simulink model "GFo_29bus"  (R2020b)
settings: Solver=ode1  StartTime=0.0  StopTime=4.5  FixedStep=Time_Step  RelTol=1e-3  EnableMultiTasking=on
PreLoadFcn:
  | Init_29bus;
InitFcn:
  | Init_29bus;
undefined symbols (not defined in the file): D1, D11, Delta, Time_Step, VSC01_Delta_P_Time_Step, VSC01_Delta_P_Value
libraries: powerlib x169, sps_avr x6, GFo_Lib x1
(part 2 of 5)

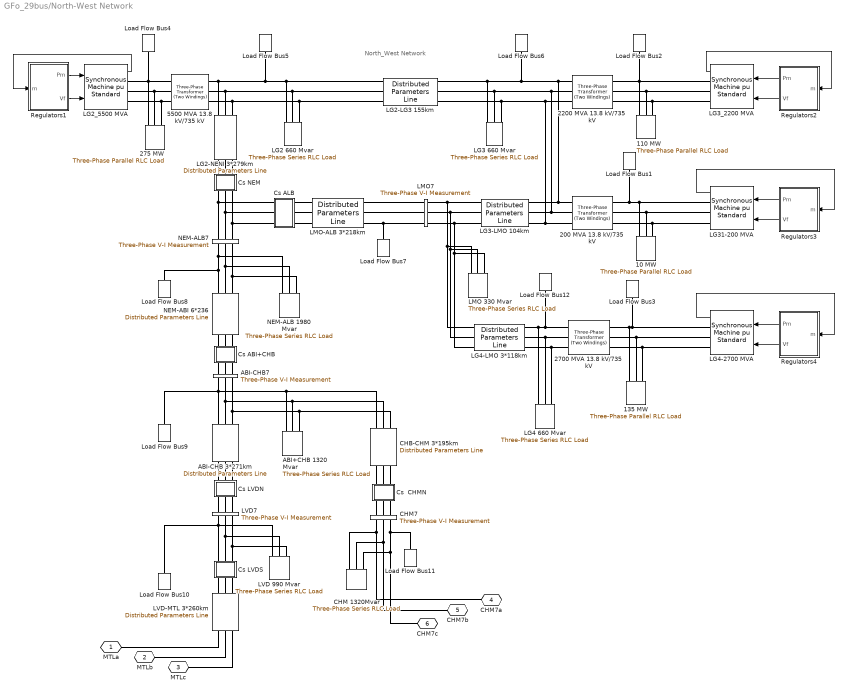
== system GFo_29bus/North-West Network ==
  note: North_West Network
  10 MW : powerlib/Elements/Three-Phase Parallel RLC Load  LConnTagsString=A|B|C  Configuration=Y (grounded)  NominalVoltage=(13800)*1  Vabc=[1e3 1e3 1e3]  Vabcp=[1e3 1e3 1e3]  NominalFrequency=60  UnbalancedPower=off  ActivePower=10000000  InductivePower=0  CapacitivePower=0  Pabc=[10e3 9e3 11e3]  QLabc=[100 90 110]  QCabc=[100 90 110]  Pabcp=[10e3 9e3 11e3]  QLabcp=[100 90 110]  QCabcp=[100 90 110]  Measurements=None  LoadType=constant PQ
  110 MW : powerlib/Elements/Three-Phase Parallel RLC Load  LConnTagsString=A|B|C  Configuration=Y (grounded)  NominalVoltage=(13800)*1  Vabc=[1e3 1e3 1e3]  Vabcp=[1e3 1e3 1e3]  NominalFrequency=60  UnbalancedPower=off  ActivePower=110000000  InductivePower=0  CapacitivePower=0  Pabc=[10e3 9e3 11e3]  QLabc=[100 90 110]  QCabc=[100 90 110]  Pabcp=[10e3 9e3 11e3]  QLabcp=[100 90 110]  QCabcp=[100 90 110]  Measurements=None  LoadType=constant PQ
  135 MW : powerlib/Elements/Three-Phase Parallel RLC Load  LConnTagsString=A|B|C  Configuration=Y (grounded)  NominalVoltage=(13800)*1  Vabc=[1e3 1e3 1e3]  Vabcp=[1e3 1e3 1e3]  NominalFrequency=60  UnbalancedPower=off  ActivePower=135000000  InductivePower=0  CapacitivePower=0  Pabc=[10e3 9e3 11e3]  QLabc=[100 90 110]  QCabc=[100 90 110]  Pabcp=[10e3 9e3 11e3]  QLabcp=[100 90 110]  QCabcp=[100 90 110]  Measurements=None  LoadType=constant PQ
  200 MVA 13.8 kV/735 kV : powerlib/Elements/Three-Phase Transformer (Two Windings)  Winding1Connection=Delta (D1)  Winding2Connection=Yg  CoreType=Three single-phase transformers  SetSaturation=off  Hysteresis=off  DataFile='basic_model'  SetInitialFlux=off  Measurements=None  UNITS=pu  NominalPower=[ 200e6 60 ]  Winding1="[ 13.8e3 0.002  0.0]"  Winding2=[ 735e3 0.002 0.12]  Rm=500  Lm=500  L0=0.5  Saturation="[ 0,0  ;  0.005,1.2  ;  1.0,1.4 ]"  InitialFluxes=[ 0.8 , -0.8 , 0.7 ]  BreakLoop=off  DiscreteSolver=Trapezoidal iterative  DataType=off  TransfoNumber=0
  2200 MVA 13.8 kV/735 kV : powerlib/Elements/Three-Phase Transformer (Two Windings)  Winding1Connection=Delta (D1)  Winding2Connection=Yg  CoreType=Three single-phase transformers  SetSaturation=off  Hysteresis=off  DataFile='basic_model'  SetInitialFlux=off  Measurements=None  UNITS=pu  NominalPower=[ 2200e6 60 ]  Winding1="[ 13.8e3 0.002  0.0]"  Winding2=[ 735e3 0.002 0.12]  Rm=500  Lm=500  L0=0.5  Saturation="[ 0,0  ;  0.005,1.2  ;  1.0,1.4 ]"  InitialFluxes=[ 0.8 , -0.8 , 0.7 ]  BreakLoop=off  DiscreteSolver=Trapezoidal iterative  DataType=off  TransfoNumber=0
  2700 MVA 13.8 kV/735 kV : powerlib/Elements/Three-Phase Transformer (Two Windings)  Winding1Connection=Delta (D1)  Winding2Connection=Yg  CoreType=Three single-phase transformers  SetSaturation=off  Hysteresis=off  DataFile='basic_model'  SetInitialFlux=off  Measurements=None  UNITS=pu  NominalPower=[ 2700e6 60 ]  Winding1="[ 13.8e3 0.002  0.0]"  Winding2=[ 735e3 0.002 0.12]  Rm=500  Lm=500  L0=0.5  Saturation="[ 0,0  ;  0.005,1.2  ;  1.0,1.4 ]"  InitialFluxes=[ 0.8 , -0.8 , 0.7 ]  BreakLoop=off  DiscreteSolver=Trapezoidal iterative  DataType=off  TransfoNumber=0
  275 MW : powerlib/Elements/Three-Phase Parallel RLC Load  LConnTagsString=A|B|C  Configuration=Y (grounded)  NominalVoltage=(13800)*1  Vabc=[1e3 1e3 1e3]  Vabcp=[1e3 1e3 1e3]  NominalFrequency=60  UnbalancedPower=off  ActivePower=275000000  InductivePower=0  CapacitivePower=0  Pabc=[10e3 9e3 11e3]  QLabc=[100 90 110]  QCabc=[100 90 110]  Pabcp=[10e3 9e3 11e3]  QLabcp=[100 90 110]  QCabcp=[100 90 110]  Measurements=None  LoadType=constant PQ
  5500 MVA 13.8 kV/735 kV : powerlib/Elements/Three-Phase Transformer (Two Windings)  Winding1Connection=Delta (D1)  Winding2Connection=Yg  CoreType=Three single-phase transformers  SetSaturation=off  Hysteresis=off  DataFile='basic_model'  SetInitialFlux=off  Measurements=None  UNITS=pu  NominalPower=[ 5500e6 60 ]  Winding1="[ 13.8e3 0.002  0.0]"  Winding2=[ 735e3 0.002 0.12]  Rm=500  Lm=500  L0=0.5  Saturation="[ 0,0  ;  0.005,1.2  ;  1.0,1.4 ]"  InitialFluxes=[ 0.8 , -0.8 , 0.7 ]  BreakLoop=off  DiscreteSolver=Trapezoidal iterative  DataType=off  TransfoNumber=0
  ABI+CHB 1320 Mvar : powerlib/Elements/Three-Phase Series RLC Load  LConnTagsString=A|B|C  Configuration=Y (grounded)  NominalVoltage=735e3  Vabc=[1e3 1e3 1e3]  Vabcp=[1e3 1e3 1e3]  NominalFrequency=60  UnbalancedPower=off  ActivePower=4400000  InductivePower=1320e6  CapacitivePower=0  Pabc=[10e3 9e3 11e3]  QLabc=[100 90 110]  QCabc=[100 90 110]  Pabcp=[10e3 9e3 11e3]  QLabcp=[100 90 110]  QCabcp=[100 90 110]  Measurements=None  LoadType=constant Z
  ABI-CHB 3*271km : powerlib/Elements/Distributed Parameters Line  Phases=3  Length=271  Frequency=60  Resistance="[0.01273  0.3864]/3"  Inductance="[0.9337e-3  4.1264e-3]/3"  Capacitance=[12.74e-9 7.751e-9]*3  x1=[-0.00156 1.39752875491723e-07 0 0;-0.00152 1.40446452432915e-07 0 0;-0.00148 1.41108093061983e-07 0 0;-0.00144 1.41737646927554e-07 0 0;-0.0014 1.42334970874506e-07 0 0;-0.00136 1.42899929076526e-07 0 0;-0.00132 1.4343239306699e-07 0 0;-0.00128 1.43932241768179e-07 0 0;-0.00124 1.44399361518809e-07 0 0;-0.0012 1.44833646099877e-07 0 0;-0.00116 1.45234996758813e-07 0 0;-0.00112 1.4560332223194e-07 0 0;-0.00108 1.45938538765221e-07 0 0;-0.00104 1.46240570133307e-07 0 0;-0.001 1.4650934765687e-07 0 0;-0.00096 1.46744810218219e-07 187826.147215716 -755236.018624843;-0.00092 1.46946904275197e-07 199193.07837809 -752317.887921003;-0.00088 1.47115583873359e-07 210514.71475221 -749228.686617163;-0.00084 1.47250810656419e-07 221788.481895596 -745969.11717106;-0.0008 1.47352553874973e-07 233011.816250821 -742539.920780675;-0.00076 1.4742079039349e-07 244182.16572844 -738941.877215697;-0.00072 1.47455504695574e-07 255296.990287309 -735175.804640203;-0.00068 1.47456688887492e-07 266353.762512174 -731242.55942662;-0.00064 1.4742434269997e-07 277349.968188381 -727143.035960991;-0.0006 1.47358473488251e-07 288283.106873586 -722878.166439598;-0.00056 1.47259096230426e-07 299150.692466336 -718448.920656993;-0.00052 1.47126233524027e-07 309950.253771385 -713856.305785471;-0.00048 1.46959915580887e-07 320679.335061623 -709101.366146047;-0.00044 1.46760180220273e-07 331335.496636489 -704185.182970991;-0.0004 1.46527072860282e-07 341916.315376735 -699108.874157963;-0.00036 1.46260646507518e-07 352419.385295425 -693873.594015808;-0.00032 1.45960961745037e-07 362842.318085035 -688480.533002086;-0.00028 1.45628086718568e-07 373182.743660531 -682930.917452362;-0.00024 1.45262097121023e-07 383438.31069831 -677226.009301355;-0.0002 1.4486307617528e-07 393606.687170866 -671367.105795981;-0.00016 1.4443111461526e-07 403685.56087708 -665355.539200373;-0.00012 1.43966310665298e-07 413672.639967986 -659192.676492932;-8e-05 1.43468770017803e-07 423565.653467925 -652879.919055492;-4e-05 1.42938605809227e-07 433362.351790939 -646418.702354656]  x2=[-0.00156 2.99200739443898e-07 0 0;-0.00152 3.00668696195938e-07 0 0;-0.00148 3.02068283479319e-07 0 0;-0.00144 3.03399183039963e-07 0 0;-0.0014 3.04661092242786e-07 0 0;-0.00136 3.05853724140519e-07 0 0;-0.00132 3.06976807538953e-07 0 0;-0.00128 3.08030087058607e-07 0 0;-0.00124 3.09013323192803e-07 0 0;-0.0012 3.09926292362122e-07 0 0;-0.00116 3.10768786965248e-07 0 0;-0.00112 3.11540615426174e-07 0 0;-0.00108 3.12241602237765e-07 0 0;-0.00104 3.12871588001663e-07 0 0;-0.001 3.13430429464539e-07 0 0;-0.00096 3.13917999550664e-07 -41952.3785136554 -761003.958677179;-0.00092 3.14334187390805e-07 -30472.3572707285 -761550.015312884;-0.00088 3.14678898347436e-07 -18985.4068765407 -761922.902042434;-0.00084 3.14952054036257e-07 -7494.13936455236 -762122.534074602;-0.0008 3.15153592344022e-07 3998.83225010076 -762148.866014787;-0.00076 3.15283467442656e-07 15490.8945647847 -762001.891875332;-0.00072 3.15341649799683e-07 26979.4343836324 -761681.64507689;-0.00068 3.15328126184936e-07 38461.839311762 -761188.198440819;-0.00064 3.15242899673569e-07 49935.4983493129 -760521.664172631;-0.0006 3.15085989645354e-07 61397.8024851645 -759682.193836469;-0.00056 3.14857431780281e-07 72846.1452902031 -758669.978320649;-0.00052 3.14557278050435e-07 84277.9235100011 -757485.24779425;-0.00048 3.14185596708187e-07 95690.5376567748 -756128.271654777;-0.00044 3.13742472270669e-07 107081.392600485 -754599.358466902;-0.0004 3.13228005500556e-07 118447.898158949 -752898.8558923;-0.00036 3.12642313383155e-07 129787.469686823 -751027.150610591;-0.00032 3.11985529099804e-07 141097.528663329 -748984.668231415;-0.00028 3.11257801997584e-07 152375.503278591 -746771.873197653;-0.00024 3.10459297555363e-07 163618.829018437 -744389.268679811;-0.0002 3.09590197346165e-07 174824.949247554 -741837.396461612;-0.00016 3.08650698995882e-07 185991.315790837 -739116.83681679;-0.00012 3.07641016138338e-07 197115.389512831 -736228.208377148;-8e-05 3.06561378366707e-07 208194.6408951 -733172.167991883;-4e-05 3.05412031181309e-07 219226.550611423 -729949.410578225]  x3=[-0.00156 3.57527130254717e-10 0 0;-0.00152 3.79613404300157e-10 0 0;-0.00148 4.01613357531105e-10 0 0;-0.00144 4.23521987347916e-10 0 0;-0.0014 4.45334311917103e-10 0 0;-0.00136 4.67045371304159e-10 0 0;-0.00132 4.88650228601409e-10 0 0;-0.00128 5.10143971050614e-10 0 0;-0.00124 5.31521711160097e-10 0 0;-0.0012 5.5277858781611e-10 0 0;-0.00116 5.73909767388214e-10 0 0;-0.00112 5.949104448284e-10 0 0;-0.00108 6.15775844763721e-10 0 0;-0.00104 6.36501222582168e-10 0 0;-0.001 6.57081865511553e-10 0 0;-0.00096 6.77513093691153e-10 139.261704598099 -1341.51413254979;-0.00092 6.97790261235871e-10 159.474777333089 -1339.26171711188;-0.00088 7.17908757292671e-10 179.651586878967 -1336.7047651088;-0.00084 7.37864007089045e-10 199.787545203237 -1333.84385796939;-0.0008 7.57651472973275e-10 219.878073562622 -1330.67964623925;-0.00076 7.77266655446258e-10 239.918603544227 -1327.21284943285;-0.00072 7.96705094184655e-10 259.904578104356 -1323.44425586989;-0.00068 8.15962369055127e-10 279.831452604746 -1319.37472249604;-0.00064 8.35034101119436e-10 299.694695845977 -1315.00517468809;-0.0006 8.53915953630177e-10 319.48979109783 -1310.33660604355;-0.00056 8.7260363301692e-10 339.212237126349 -1305.37007815465;-0.00052 8.91092889862529e-10 358.857549217388 -1300.10672036701;-0.00048 9.0937951986944e-10 378.42126019639 -1294.5477295228;-0.00044 9.27459364815689e-10 397.89892144419 -1288.6943696886;-0.0004 9.45328313500447e-10 417.286103908588 -1282.54797186797;-0.00036 9.62982302678879e-10 436.578399111478 -1276.10993369875;-0.00032 9.80417317986088e-10 455.771420151303 -1269.38171913531;-0.00028 9.97629394849945e-10 474.860802700591 -1262.36485811562;-0.00024 1.0146146193926e-09 493.842205998369 -1255.06094621337;-0.0002 1.03136912932048e-09 512.711313837218 -1247.47164427514;-0.00016 1.04788911480249e-09 531.463835544733 -1239.59867804273;-0.00012 1.06417081933641e-09 550.095506959195 -1231.44383776078;-8e-05 1.08021054060303e-09 568.602091399196 -1223.00897776964;-4e-05 1.09600463130805e-09 586.979380627029 -1214.29601608374]  x4=[-0.00156 1.09221564098943e-09 0 0;-0.00152 1.08563764232773e-09 0 0;-0.00148 1.07881277902829e-09 0 0;-0.00144 1.0717426030062e-09 0 0;-0.0014 1.06442872195849e-09 0 0;-0.00136 1.05687279899865e-09 0 0;-0.00132 1.0490765522784e-09 0 0;-0.00128 1.04104175459702e-09 0 0;-0.00124 1.0327702329982e-09 0 0;-0.0012 1.02426386835463e-09 0 0;-0.00116 1.01552459494027e-09 0 0;-0.00112 1.00655439999053e-09 0 0;-0.00108 9.97355323250386e-10 0 0;-0.00104 9.87929456510564e-10 0 0;-0.001 9.78278943131873e-10 0 0;-0.00096 9.68405977557831e-10 -1510.55195138334 -15585.3803111024;-0.00092 9.58312804815671e-10 -1275.36683491454 -15606.3854409047;-0.00088 9.48001720005832e-10 -1039.89171102577 -15623.8418132415;-0.00084 9.37475067780084e-10 -804.180124729557 -15637.7454586843;-0.0008 9.26735241808363e-10 -568.285674807936 -15648.0932156639;-0.00076 9.15784684234478e-10 -332.262001624548 -15654.8827311897;-0.00072 9.0462588512079e-10 -96.1627749272983 -15658.1124613844;-0.00068 8.93261381881987e-10 139.958318355698 -15657.7816718352;-0.00064 8.81693758708102e-10 376.04758632405 -15653.8904377607;-0.0006 8.69925645976889e-10 612.051344314168 -15646.4396439941;-0.00056 8.57959719655701e-10 847.915927106694 -15635.4309847816;-0.00052 8.45798700692993e-10 1083.58770112951 -15620.8669633974;-0.00048 8.33445354399604e-10 1319.01307665356 -15602.7508915744;-0.00044 8.20902489819951e-10 1554.13851997865 -15581.0868887509;-0.0004 8.08172959093275e-10 1788.91056560663 -15555.8798811346;-0.00036 7.95259656805089e-10 2023.27582839889 -15527.1356005815;-0.00032 7.82165519328971e-10 2257.18101571576 -15494.8605832931;-0.00028 7.68893524158867e-10 2490.57293953476 -15459.0621683301;-0.00024 7.55446689232024e-10 2723.39852854509 -15419.7484959432;-0.0002 7.41828072242744e-10 2955.60484021562 -15376.9285057226;-0.00016 7.2804076994709e-10 3187.13907283354 -15330.6119345649;-0.00012 7.14087917458705e-10 3417.94857751101 -15280.8093144587;-8e-05 6.99972687535923e-10 3647.98087015709 -15227.5319700906;-4e-05 6.85698289860302e-10 3877.18364341214 -15170.792016269]  x5=0.00153261764655846  V1=ones(3,3)  V2=ones(3,3)  I1=ones(3,3)  I2=ones(3,3)  nHarmo=1  Measurements=None  Decoupling=off  VsMag0=0  VrMag0=0  VsAngle0=0  VrAngle0=0  IsMag0=0  IrMag0=0  IsAngle0=0  IrAngle0=0
      settings: AttributesFormatString=\n
  ABI-CHB7 : powerlib/Measurements/Three-Phase V-I Measurement  VoltageMeasurement=no  SetLabelV=on  LabelV=Vabc_ABI7  Vpu=on  VpuLL=off  CurrentMeasurement=no  SetLabelI=off  LabelI=A1  Ipu=off  Pbase=100e6  Vbase=500e3  OutputType=Magnitude  PhasorSimulation=off  PSBequivalent=0
  CHB-CHM 3*195km : powerlib/Elements/Distributed Parameters Line  Phases=3  Length=195  Frequency=60  Resistance="[0.01273  0.3864]/3"  Inductance="[0.9337e-3  4.1264e-3]/3"  Capacitance=[12.74e-9 7.751e-9]*3  x1=[-0.00112 1.45810315855676e-07 0 0;-0.00108 1.46144986641095e-07 0 0;-0.00104 1.46446425316851e-07 0 0;-0.001 1.46714563338391e-07 0 0;-0.00096 1.4694933973344e-07 0 0;-0.00092 1.47150701115871e-07 0 0;-0.00088 1.47318601697842e-07 0 0;-0.00084 1.47453003300208e-07 0 0;-0.0008 1.47553875361205e-07 0 0;-0.00076 1.47621194943394e-07 0 0;-0.00072 1.47654946738885e-07 0 0;-0.00068 1.47655123072809e-07 266353.762512174 -731242.55942662;-0.00064 1.4762172390507e-07 277349.968188381 -727143.035960991;-0.0006 1.4755475683035e-07 288283.106873586 -722878.166439599;-0.00056 1.47454237076385e-07 299150.692466336 -718448.920656994;-0.00052 1.473201875005e-07 309950.253771385 -713856.305785471;-0.00048 1.47152638584413e-07 320679.335061623 -709101.366146047;-0.00044 1.46951628427302e-07 331335.496636489 -704185.182970992;-0.0004 1.46717202737144e-07 341916.315376735 -699108.874157963;-0.00036 1.46449414820318e-07 352419.385295425 -693873.594015809;-0.00032 1.46148325569488e-07 362842.318085035 -688480.533002086;-0.00028 1.45814003449753e-07 373182.743660531 -682930.917452362;-0.00024 1.4544652448308e-07 383438.31069831 -677226.009301355;-0.0002 1.45045972231017e-07 393606.687170866 -671367.105795982;-0.00016 1.44612437775692e-07 403685.56087708 -665355.539200373;-0.00012 1.44146019699101e-07 413672.639967986 -659192.676492932;-8e-05 1.43646824060693e-07 423565.653467925 -652879.919055493;-4e-05 1.43114964373251e-07 433362.351790939 -646418.702354656]  x2=[-0.00112 1.02653671848885e-07 0 0;-0.00108 1.02818285588003e-07 0 0;-0.00104 1.02959519335645e-07 0 0;-0.001 1.03077340976476e-07 0 0;-0.00096 1.03171723718869e-07 0 0;-0.00092 1.03242646101004e-07 0 0;-0.00088 1.03290091995742e-07 0 0;-0.00084 1.03314050614296e-07 0 0;-0.0008 1.03314516508683e-07 0 0;-0.00076 1.03291489572962e-07 0 0;-0.00072 1.0324497504326e-07 0 0;-0.00068 1.03174983496581e-07 189059.279163622 -739106.876621779;-0.00064 1.03081530848397e-07 200182.85637729 -736171.980405194;-0.0006 1.02964638349035e-07 211260.913735721 -733069.685028741;-0.00056 1.02824332578842e-07 222290.932184205 -729800.695927637;-0.00052 1.0266064544214e-07 233270.403591666 -726365.756441812;-0.00048 1.02473614159972e-07 244196.831320988 -722765.647646883;-0.00044 1.02263281261639e-07 255067.730796732 -719001.188176545;-0.0004 1.02029694575028e-07 265880.630070103 -715073.234036418;-0.00036 1.01772907215738e-07 276633.070381053 -710982.6784094;-0.00032 1.01492977574998e-07 287322.60671738 -706730.451452565;-0.00028 1.01189969306396e-07 297946.808370705 -702317.520085654;-0.00024 1.00863951311399e-07 308503.25948919 -697744.887771204;-0.0002 1.00514997723688e-07 318989.559626885 -693013.59428637;-0.00016 1.00143187892299e-07 329403.324289571 -688124.71548649;-0.00012 9.97486063635805e-08 339742.185476966 -683079.363060443;-8e-05 9.93313428619707e-08 350003.792221196 -677878.684277862;-4e-05 9.88914922695912e-08 360185.811121378 -672523.861728252]  x3=[-0.00112 5.46806558992984e-10 0 0;-0.00108 5.43566628750611e-10 0 0;-0.00104 5.40203096144379e-10 0 0;-0.001 5.36716726012596e-10 0 0;-0.00096 5.33108311125766e-10 0 0;-0.00092 5.29378672006317e-10 0 0;-0.00088 5.2552865674202e-10 0 0;-0.00084 5.21559140793147e-10 0 0;-0.0008 5.17471026793391e-10 0 0;-0.00076 5.13265244344623e-10 0 0;-0.00072 5.08942749805502e-10 0 0;-0.00068 5.0450452607401e-10 1436.68883540451 -5039.58498648989;-0.00064 4.99951582363951e-10 1512.51770856541 -5017.34797480586;-0.0006 4.95284953975461e-10 1588.00264824277 -4993.97006146011;-0.00056 4.90505702059593e-10 1663.12648981228 -4969.45656238856;-0.00052 4.85614913377017e-10 1737.87215076019 -4943.81305174949;-0.00048 4.80613700050904e-10 1812.2226345678 -4917.04536065607;-0.00044 4.75503199314036e-10 1886.16103457624 -4889.15957585044;-0.0004 4.70284573250208e-10 1959.67053783099 -4860.16203831958;-0.00036 4.64959008529985e-10 2032.7344289049 -4830.05934185345;-0.00032 4.59527716140858e-10 2105.33609369925 -4798.85833154564;-0.00028 4.53991931111878e-10 2177.45902322152 -4766.56610223683;-0.00024 4.48352912232824e-10 2249.08681733953 -4733.18999690149;-0.0002 4.42611941767958e-10 2320.20318851057 -4698.73760497815;-0.00016 4.36770325164458e-10 2390.79196548512 -4663.21676064362;-0.00012 4.30829390755561e-10 2460.83709698404 -4626.63554103159;-8e-05 4.24790489458522e-10 2530.32265534845 -4589.00226439593;-4e-05 4.18654994467416e-10 2599.23284016162 -4550.32548821922]  x4=[-0.00112 3.66592185990391e-10 0 0;-0.00108 3.74745086886299e-10 0 0;-0.00104 3.82812773981113e-10 0 0;-0.001 3.90793412752361e-10 0 0;-0.00096 3.98685188471607e-10 0 0;-0.00092 4.0648630661711e-10 0 0;-0.00088 4.14194993281876e-10 0 0;-0.00084 4.21809495577036e-10 0 0;-0.0008 4.29328082030432e-10 0 0;-0.00076 4.36749042980341e-10 0 0;-0.00072 4.44070690964241e-10 0 0;-0.00068 4.51291361102517e-10 1508.00651437075 -11782.2938614844;-0.00064 4.5840941147705e-10 1685.50172841415 -11758.2144968013;-0.0006 4.65423223504567e-10 1862.61367389965 -11731.4614155401;-0.00056 4.72331202304699e-10 2039.3020770982 -11702.0407011208;-0.00052 4.79131777062637e-10 2215.52676059061 -11669.9590435602;-0.00048 4.85823401386327e-10 2391.24765240356 -11635.2237379506;-0.00044 4.92404553658105e-10 2566.42479512158 -11597.8426828008;-0.0004 4.98873737380697e-10 2741.01835497311 -11557.8243782405;-0.00036 5.05229481517512e-10 2914.98863088824 -11515.177924087;-0.00032 5.11470340827144e-10 3088.29606352651 -11469.9130177763;-0.00028 5.17594896192004e-10 3260.90124427226 -11422.0399521576;-0.00024 5.23601754941019e-10 3432.76492419587 -11371.5696131533;-0.0002 5.29489551166309e-10 3603.84802297863 -11318.5134772832;-0.00016 5.35256946033787e-10 3774.11163779923 -11262.883609055;-0.00012 5.40902628087596e-10 3943.51705217994 -11204.6926582211;-8e-05 5.46425313548324e-10 4112.02574479043 -11143.9538569019;-4e-05 5.51823746604922e-10 4279.59939820715 -11080.681016577]  x5=0.0011028060556417  V1=ones(3,3)  V2=ones(3,3)  I1=ones(3,3)  I2=ones(3,3)  nHarmo=1  Measurements=None  Decoupling=off  VsMag0=0  VrMag0=0  VsAngle0=0  VrAngle0=0  IsMag0=0  IrMag0=0  IsAngle0=0  IrAngle0=0
      settings: AttributesFormatString=\n
  CHM 1320Mvar : powerlib/Elements/Three-Phase Series RLC Load  LConnTagsString=A|B|C  Configuration=Y (grounded)  NominalVoltage=735e3  Vabc=[1e3 1e3 1e3]  Vabcp=[1e3 1e3 1e3]  NominalFrequency=60  UnbalancedPower=off  ActivePower=4400000  InductivePower=1320e6  CapacitivePower=0  Pabc=[10e3 9e3 11e3]  QLabc=[100 90 110]  QCabc=[100 90 110]  Pabcp=[10e3 9e3 11e3]  QLabcp=[100 90 110]  QCabcp=[100 90 110]  Measurements=None  LoadType=constant Z
  CHM7 : powerlib/Measurements/Three-Phase V-I Measurement  VoltageMeasurement=no  SetLabelV=on  LabelV=Vabc_CHM7  Vpu=on  VpuLL=off  CurrentMeasurement=no  SetLabelI=off  LabelI=A1  Ipu=off  Pbase=100e6  Vbase=735e3  OutputType=Magnitude  PhasorSimulation=off  PSBequivalent=0
  "Cs  CHMN " : Subsystem  mask{Xc=25/3}
      mask prompts: Xc "Condensator Reactance at  60Hz  (ohm):"
      mask help: Series Compensation
      mask init:
      | Cs=1/Xc/(2*pi*60);
      mask Display: disp('Cs')
  "Cs ABI+CHB " : Subsystem  mask{Xc=25/6}
      mask prompts: Xc "Condensator Reactance at  60Hz  (ohm):"
      mask help: Series Compensation
      mask init:
      | Cs=1/Xc/(2*pi*60);
      mask Display: disp('Cs')
  Cs ALB : Subsystem  mask{Xc=16/3}
      mask prompts: Xc "Reactance @ 60Hz du condensateur (ohm):"
      mask init:
      | Cs=1/Xc/(2*pi*60);
      mask Display: disp('Cs')
  "Cs LVDN " : Subsystem  mask{Xc=34/3}
      mask prompts: Xc "Condensator Reactance at  60Hz  (ohm):"
      mask help: Series Compensation
      mask init:
      | Cs=1/Xc/(2*pi*60);
      mask Display: disp('Cs')
  "Cs LVDS " : Subsystem  mask{Xc=34/3}
      mask prompts: Xc "Condensator Reactance at  60Hz  (ohm):"
      mask help: Series Compensation
      mask init:
      | Cs=1/Xc/(2*pi*60);
      mask Display: disp('Cs')
  "Cs NEM " : Subsystem  mask{Xc=16/3}
      mask prompts: Xc "Condensator Reactance at  60Hz  (ohm):"
      mask help: Series Compensation
      mask init:
      | Cs=1/Xc/(2*pi*60);
      mask Display: disp('Cs')
  LG2 660 Mvar : powerlib/Elements/Three-Phase Series RLC Load  LConnTagsString=A|B|C  Configuration=Y (grounded)  NominalVoltage=735e3  Vabc=[1e3 1e3 1e3]  Vabcp=[1e3 1e3 1e3]  NominalFrequency=60  UnbalancedPower=off  ActivePower=2200000  InductivePower=660e6  CapacitivePower=0  Pabc=[10e3 9e3 11e3]  QLabc=[100 90 110]  QCabc=[100 90 110]  Pabcp=[10e3 9e3 11e3]  QLabcp=[100 90 110]  QCabcp=[100 90 110]  Measurements=None  LoadType=constant Z
  LG2-LG3 155km : powerlib/Elements/Distributed Parameters Line  Phases=3  Length=155  Frequency=60  Resistance="[0.01273  0.3864]"  Inductance="[0.9337e-3  4.1264e-3]"  Capacitance=[12.74e-9 7.751e-9]  x1=[-0.00088 8.27904700189463e-09 432972.643007168 -601762.460463716;-0.00084 8.1824988858554e-09 441997.469609916 -595165.210790078;-0.0008 8.08409014013239e-09 450921.789799698 -588432.625679992;-0.00076 7.98384314202574e-09 459743.574263063 -581566.236065254;-0.00072 7.88178068683832e-09 468460.817002301 -574567.603303648;-0.00068 7.7779259826923e-09 477071.535791587 -567438.318823911;-0.00064 7.67230264525179e-09 485573.772627723 -560180.003763853;-0.0006 7.56493469235287e-09 493965.594175373 -552794.308601725;-0.00056 7.45584653854213e-09 502245.092206687 -545282.912780917;-0.00052 7.345062989525e-09 510410.384035209 -537647.524328061;-0.00048 7.23260923652519e-09 518459.612943993 -529889.879464649;-0.00044 7.11851085055635e-09 526390.9486078 -522011.742212222;-0.0004 7.00279377660752e-09 534202.587509295 -514014.903991253;-0.00036 6.88548432774341e-09 541892.753349157 -505901.183213792;-0.00032 6.76660917912106e-09 549459.697449992 -497672.424869975;-0.00028 6.64619536192413e-09 556901.699153965 -489330.500108486;-0.00024 6.52427025721625e-09 564217.066214066 -480877.305811079;-0.0002 6.40086158971478e-09 571404.135178912 -472314.76416124;-0.00016 6.27599742148649e-09 578461.271770996 -463644.8222071;-0.00012 6.14970614556646e-09 585386.871258318 -454869.451418693;-8e-05 6.02201647950173e-09 592179.358819277 -445990.64723966;-4e-05 5.89295745882122e-09 598837.189900778 -437010.428633504]  x2=[-0.00088 2.7409355673421e-09 445028.999861563 -584528.468417923;-0.00084 2.64624629672137e-09 453792.581408512 -577751.376045215;-0.0008 2.55095529251302e-09 462452.97443579 -570842.90799191;-0.00076 2.45508422306966e-09 471008.209644705 -563804.635184068;-0.00072 2.35865488864571e-09 479456.341648548 -556638.158064228;-0.00068 2.26168921644027e-09 487795.449414957 -549345.106227488;-0.00064 2.16420925561097e-09 496023.636702737 -541927.138050943;-0.0006 2.0662371722603e-09 504139.032493056 -534385.940316585;-0.00056 1.96779524439513e-09 512139.791414897 -526723.227827747;-0.00052 1.86890585686093e-09 520024.094164675 -518940.743019169;-0.00048 1.76959149625163e-09 527790.147919937 -511040.255560782;-0.00044 1.66987474579639e-09 535436.18674703 -503023.561955305;-0.0004 1.56977828022435e-09 542960.472002662 -494892.485129729;-0.00036 1.46932486060857e-09 550361.292729253 -486648.874020806;-0.00032 1.36853732919041e-09 557636.96604399 -478294.603154611;-0.00028 1.26743860418535e-09 564785.837521505 -469831.572220297;-0.00024 1.16605167457163e-09 571806.281570074 -461261.705638114;-0.0002 1.06439959486271e-09 578696.701801261 -452586.952121821;-0.00016 9.62505479864911e-10 585455.531392926 -443809.284235559;-0.00012 8.60392499421284e-10 592081.233445506 -434930.69794531;-8e-05 7.58083873142997e-10 598572.301331491 -425953.21216503;-4e-05 6.55602865129395e-10 604927.259038022 -416878.868297569]  x3=[-0.00088 7.27991996063612e-12 1691.0601492433 -2581.83555988018;-0.00084 6.86444585434417e-12 1729.79962719017 -2556.0423915541;-0.0008 6.44741083226141e-12 1768.14576361897 -2529.66800123056;-0.00076 6.02890972455549e-12 1806.08983894897 -2502.71838621846;-0.00072 5.60903769476932e-12 1843.62322502464 -2475.19967462786;-0.00068 5.18789021818163e-12 1880.73738707768 -2447.11812397646;-0.00064 4.76556306009679e-12 1917.42388566768 -2418.48011976672;-0.0006 4.34215225406855e-12 1953.67437860124 -2389.29217403383;-0.00056 3.91775408006286e-12 1989.48062282887 -2359.56092386494;-0.00052 3.49246504256463e-12 2024.83447631943 -2329.29312988995;-0.00048 3.06638184863347e-12 2059.7278999115 -2298.49567474419;-0.00044 2.63960138591327e-12 2094.15295914146 -2267.17556150338;-0.0004 2.21222070060087e-12 2128.10182604773 -2235.33991209117;-0.00036 1.78433697537853e-12 2161.56678095071 -2202.99596565971;-0.00032 1.35604750731546e-12 2194.54021420827 -2170.15107694348;-0.00028 9.2744968574328e-13 2227.01462794603 -2136.81271458693;-0.00024 4.98640970110547e-13 2258.98263776235 -2102.98845944618;-0.0002 6.97188678213079e-14 2290.43697440747 -2068.68600286516;-0.00016 -3.59219087937244e-13 2321.37048543651 -2033.91314492666;-0.00012 -7.88075360372972e-13 2351.7761368358 -1998.67779267874;-8e-05 -1.21675243126782e-12 2381.64701462243 -1962.98795833662;-4e-05 -1.64515282315263e-12 2410.97632641638 -1926.85175746086]  x4=[-0.00088 1.00066401297176e-11 1092.96989342867 -2102.93040181918;-0.00084 1.02141033117926e-11 1124.5560468815 -2086.21026082815;-0.0008 1.04192438948573e-11 1155.88648598704 -2069.01573361452;-0.00076 1.06220152317119e-11 1186.95408647359 -2051.35073006549;-0.00072 1.08223712139033e-11 1217.75178383675 -2033.21926705055;-0.00068 1.10202662822087e-11 1248.2725749457 -2014.62546750801;-0.00064 1.12156554369963e-11 1278.50951963575 -1995.57355950756;-0.0006 1.14084942484572e-11 1308.45574228643 -1976.06787528876;-0.00056 1.15987388667087e-11 1338.10443338496 -1956.11285027601;-0.00052 1.17863460317652e-11 1367.44885107466 -1935.7130220699;-0.00048 1.19712730833751e-11 1396.482322688 -1914.87302941546;-0.00044 1.21534779707218e-11 1425.19824626391 -1893.59761114728;-0.0004 1.2332919261985e-11 1453.59009204901 -1871.89160511202;-0.00036 1.25095561537627e-11 1481.6514039824 -1849.75994706827;-0.00032 1.26833484803488e-11 1509.37580116375 -1827.2076695642;-0.00028 1.2854256722867e-11 1536.75697930421 -1804.23990079324;-0.00024 1.30222420182568e-11 1563.78871216001 -1780.86186342794;-0.0002 1.31872661681107e-11 1590.4648529482 -1757.0788734324;-0.00016 1.33492916473601e-11 1616.77933574442 -1732.89633885344;-0.00012 1.35082816128082e-11 1642.7261768622 -1708.31975859089;-8e-05 1.36641999115081e-11 1668.29947621362 -1683.35472114715;-4e-05 1.38170110889832e-11 1693.49341865096 -1658.00690335646]  x5=0.000876589428843401  V1=ones(3,3)  V2=ones(3,3)  I1=ones(3,3)  I2=ones(3,3)  nHarmo=1  Measurements=None  Decoupling=off  VsMag0=0  VrMag0=0  VsAngle0=0  VrAngle0=0  IsMag0=0  IrMag0=0  IsAngle0=0  IrAngle0=0
      settings: AttributesFormatString=\n
  LG2-NENI 3*279km : powerlib/Elements/Distributed Parameters Line  Phases=3  Length=279  Frequency=60  Resistance="[0.01273  0.3864]/3"  Inductance="[0.9337e-3  4.1264e-3]/3"  Capacitance=[12.74e-9 7.751e-9]*3  x1=[-0.0016 9.6758636722634e-09 0 0;-0.00156 9.61612844832559e-09 0 0;-0.00152 9.55420659970459e-09 0 0;-0.00148 9.49011220689479e-09 0 0;-0.00144 9.42385984440838e-09 0 0;-0.0014 9.35546457746126e-09 0 0;-0.00136 9.28494195854731e-09 0 0;-0.00132 9.21230802390192e-09 0 0;-0.00128 9.13757928985545e-09 0 0;-0.00124 9.0607727490776e-09 0 0;-0.0012 8.98190586671339e-09 0 0;-0.00116 8.90099657641174e-09 0 0;-0.00112 8.81806327624754e-09 0 0;-0.00108 8.73312482453806e-09 0 0;-0.00104 8.64620053555475e-09 0 0;-0.001 8.5573101751313e-09 405315.757865055 -620727.351199328;-0.00096 8.46647395616913e-09 414629.701621394 -614544.98398615;-0.00092 8.37371253404109e-09 423849.362159198 -608222.874543223;-0.00088 8.27904700189463e-09 432972.643007168 -601762.460463716;-0.00084 8.1824988858554e-09 441997.469609916 -595165.210790078;-0.0008 8.08409014013239e-09 450921.789799698 -588432.625679992;-0.00076 7.98384314202574e-09 459743.574263063 -581566.236065254;-0.00072 7.88178068683832e-09 468460.817002301 -574567.603303648;-0.00068 7.7779259826923e-09 477071.535791587 -567438.318823911;-0.00064 7.67230264525179e-09 485573.772627723 -560180.003763853;-0.0006 7.56493469235287e-09 493965.594175373 -552794.308601725;-0.00056 7.45584653854213e-09 502245.092206687 -545282.912780917;-0.00052 7.345062989525e-09 510410.384035209 -537647.524328061;-0.00048 7.23260923652519e-09 518459.612943993 -529889.879464649;-0.00044 7.11851085055635e-09 526390.9486078 -522011.742212222;-0.0004 7.00279377660752e-09 534202.587509295 -514014.903991253;-0.00036 6.88548432774341e-09 541892.753349157 -505901.183213792;-0.00032 6.76660917912106e-09 549459.697449992 -497672.424869975;-0.00028 6.64619536192413e-09 556901.699153965 -489330.500108486;-0.00024 6.52427025721625e-09 564217.066214066 -480877.305811079;-0.0002 6.40086158971478e-09 571404.135178912 -472314.76416124;-0.00016 6.27599742148649e-09 578461.271770996 -463644.8222071;-0.00012 6.14970614556646e-09 585386.871258318 -454869.451418693;-8e-05 6.02201647950173e-09 592179.358819277 -445990.64723966;-4e-05 5.89295745882122e-09 598837.189900778 -437010.428633504]  x2=[-0.0016 8.5354922288783e-08 0 0;-0.00156 8.57697620739079e-08 0 0;-0.00152 8.61650985547841e-08 0 0;-0.00148 8.65408418353052e-08 0 0;-0.00144 8.68969064746893e-08 0 0;-0.0014 8.72332115069081e-08 0 0;-0.00136 8.75496804590974e-08 0 0;-0.00132 8.78462413689465e-08 0 0;-0.00128 8.81228268010621e-08 0 0;-0.00124 8.83793738623021e-08 0 0;-0.0012 8.8615824216077e-08 0 0;-0.00116 8.88321240956154e-08 0 0;-0.00112 8.90282243161902e-08 0 0;-0.00108 8.92040802863021e-08 0 0;-0.00104 8.93596520178202e-08 0 0;-0.001 8.94949041350743e-08 243862.200065096 -727663.3089743;-0.00096 8.96098058828992e-08 254806.991474155 -723903.345217886;-0.00092 8.97043311336284e-08 265693.841970715 -719978.772083446;-0.00088 8.9778458393035e-08 276520.275978857 -715890.481985067;-0.00084 8.98321708052195e-08 287283.831660851 -711639.404564661;-0.0008 8.98654561564425e-08 297982.061476955 -707226.506480574;-0.00076 8.98783068779022e-08 308612.532741968 -702652.791187774;-0.00072 8.98707200474555e-08 319172.828178396 -697919.298709679;-0.00068 8.9842697390282e-08 329660.546466125 -693027.105401656;-0.00064 8.97942452784923e-08 340073.30278846 -687977.323706276;-0.0006 8.9725374729679e-08 350408.729374407 -682771.101900349;-0.00056 8.96361014044108e-08 360664.476037091 -677409.623833817;-0.00052 8.9526445602672e-08 370838.210708163 -671894.108660558;-0.00048 8.93964322592464e-08 380927.619968091 -666225.810561157;-0.00044 8.9246090938047e-08 390930.409572219 -660406.01845772;-0.0004 8.90754558253938e-08 400844.304972451 -654436.055720786;-0.00036 8.888456572224e-08 410667.051834466 -648317.279868397;-0.00032 8.86734640353487e-08 420396.416550335 -642051.082257416;-0.00028 8.84421987674232e-08 430030.186746425 -635638.887767142;-0.00024 8.81908225061911e-08 439566.171786472 -629082.154475306;-0.0002 8.79193924124462e-08 449002.203269711 -622382.373326516;-0.00016 8.76279702070514e-08 458336.135523957 -615541.067793229;-0.00012 8.73166221569029e-08 467565.846093507 -608559.793529326;-8e-05 8.69854190598624e-08 476689.236221772 -601440.13801637;-4e-05 8.66344362286579e-08 485704.231328513 -594183.720202628]  x3=[-0.0016 -5.46808078159071e-11 0 0;-0.00156 -4.6617977209578e-11 0 0;-0.00152 -3.85445460772478e-11 0 0;-0.00148 -3.04623502475336e-11 0 0;-0.00144 -2.23732275420693e-11 0 0;-0.0014 -1.42790173576004e-11 0 0;-0.00136 -6.18156024772144e-12 0 0;-0.00132 1.91730249565047e-12 0 0;-0.00128 1.00157292609689e-11 0 0;-0.00124 1.81118785358254e-11 0 0;-0.0012 2.6203909325693e-11 0 0;-0.00116 3.42899815725528e-11 0 0;-0.00112 4.23682565733073e-11 0 0;-0.00108 5.04368973978852e-11 0 0;-0.00104 5.84940693069441e-11 0 0;-0.001 6.65379401690741e-11 -295.463539849934 -2742.8851540493;-0.00096 7.45666808774083e-11 -254.069695765629 -2747.02858681015;-0.00092 8.25784657655467e-11 -212.61807842351 -2750.54736895973;-0.00088 9.05714730226964e-11 -171.118113563898 -2753.44070035731;-0.00084 9.85438851079358e-11 -129.579237920922 -2755.7079230843;-0.0008 1.06493889163508e-10 -88.0108970766856 -2757.34852159379;-0.00076 1.14419677427048e-10 -46.4225433134278 -2758.36212282783;-0.00072 1.22319447642655e-10 -4.82363346415175 -2758.74849630224;-0.00068 1.30191403470706e-10 36.7763732377769 -2758.50755415902;-0.00064 1.38033754896331e-10 78.3680173095774 -2757.63935118635;-0.0006 1.45844718636444e-10 119.941841170059 -2756.14408480608;-0.00056 1.53622518545251e-10 161.488391290192 -2754.0220950289;-0.00052 1.61365386018125e-10 202.998220342763 -2751.27386437699;-0.00048 1.69071560393774e-10 244.46188935061 -2747.9000177743;-0.00044 1.76739289354601e-10 285.869969832968 -2743.90132240444;-0.0004 1.84366829325163e-10 327.213045949423 -2739.27868753627;-0.00036 1.91952445868649e-10 368.481716640995 -2734.03316431708;-0.00032 1.99494414081271e-10 409.666597767854 -2728.16594553363;-0.00028 2.06991018984498e-10 450.758324243195 -2721.67836534086;-0.00024 2.14440555915022e-10 491.747552162777 -2714.57189895857;-0.0002 2.21841330912388e-10 532.624960929647 -2706.84816233592;-0.00016 2.29191661104182e-10 573.381255373564 -2698.50891178403;-0.00012 2.36489875088706e-10 614.007167864638 -2689.55604357655;-8e-05 2.43734313315037e-10 654.493460420713 -2679.9915935185;-4e-05 2.50923328460395e-10 694.830926807998 -2669.81773648334]  x4=[-0.0016 3.75262064378135e-10 0 0;-0.00156 3.7019294113375e-10 0 0;-0.00152 3.65039639206959e-10 0 0;-0.00148 3.5980333041418e-10 0 0;-0.00144 3.54485205446877e-10 0 0;-0.0014 3.49086473600805e-10 0 0;-0.00136 3.4360836250103e-10 0 0;-0.00132 3.38052117822774e-10 0 0;-0.00128 3.32419003008163e-10 0 0;-0.00124 3.26710298978928e-10 0 0;-0.0012 3.20927303845134e-10 0 0;-0.00116 3.15071332610005e-10 0 0;-0.00112 3.091437168709e-10 0 0;-0.00108 3.0314580451652e-10 0 0;-0.00104 2.97078959420411e-10 0 0;-0.001 2.9094456113083e-10 4695.72941749195 -13362.2957077437;-0.00096 2.84744004557047e-10 4896.68712230063 -13289.9688778751;-0.00092 2.78478699652156e-10 5096.53136268494 -13214.6200236916;-0.00088 2.72150071092461e-10 5295.21669578799 -13136.2662788727;-0.00084 2.65759557953522e-10 5492.69794227842 -13054.9254603843;-0.0008 2.59308613382918e-10 5688.93019662378 -12970.6160644271;-0.00076 2.52798704269812e-10 5883.86883730168 -12883.3572622307;-0.00072 2.46231310911399e-10 6077.4695369463 -12793.1688956942;-0.00068 2.39607926676293e-10 6269.68827242808 -12700.0714728744;-0.00064 2.32930057664951e-10 6460.4813348642 -12604.0861633224;-0.0006 2.26199222367199e-10 6649.80533955759 -12505.2347932699;-0.00056 2.19416951316941e-10 6837.61723586224 -12403.539840666;-0.00052 2.12584786744124e-10 7023.87431697256 -12299.0244300658;-0.00048 2.05704282224054e-10 7208.53422963451 -12191.7123273726;-0.00044 1.98777002324125e-10 7391.5549837764 -12081.6279344329;-0.0004 1.91804522248048e-10 7572.89496205703 -11968.7962834885;-0.00036 1.84788427477662e-10 7752.51292932915 -11853.2430314837;-0.00032 1.77730313412416e-10 7930.36804201597 -11734.9944542315;-0.00028 1.70631785006581e-10 8106.41985739861 -11614.0774404388;-0.00024 1.63494456404302e-10 8280.62834281247 -11490.5194855916;-0.0002 1.56319950572552e-10 8452.95388475027 -11364.3486857034;-0.00016 1.49109898932088e-10 8623.35729786984 -11235.5937309261;-0.00012 1.41865940986475e-10 8791.79983390456 -11104.283899026;-8e-05 1.34589723949282e-10 8958.24319047429 -10970.4490487265;-4e-05 1.27282902369515e-10 9122.6495197951 -10834.1196129185]  x5=0.00157786097191812  V1=ones(3,3)  V2=ones(3,3)  I1=ones(3,3)  I2=ones(3,3)  nHarmo=1  Measurements=None  Decoupling=off  VsMag0=0  VrMag0=0  VsAngle0=0  VrAngle0=0  IsMag0=0  IrMag0=0  IsAngle0=0  IrAngle0=0
      settings: AttributesFormatString=\n
  LG2_5500 MVA : powerlib/Machines/Synchronous Machine pu Standard  PresetModel=No  MechanicalLoad=Mechanical power Pm  ShowDetailedParameters=on  RotorType=Salient-pole  Units=per unit standard parameters  MeasurementBus=off  NominalParameters="[5500E6  13800   60 ]"  Reactances1=[ 31 32 33 34 35 36 37 ]  Reactances2=[ 1.305, 0.296, 0.252, 0.474, 0.243, 0.18 ]  dAxisTimeConstants=Short-circuit  qAxisTimeConstants=Open-circuit  TimeConstants1=[]  TimeConstants2=[]  TimeConstants3=[]  TimeConstants4=[]  TimeConstants5=[ 1.01, 0.053, 0.1 ]  TimeConstants6=[]  TimeConstants7=[]  TimeConstants8=[]  StatorResistance=2.8544e-3  Mechanical="[ 4.1  0  32]"  PolePairs=32  InitialConditions=[0 -68.2322 0.822292 0.822292 0.822292 4.1842 -115.816 124.184 1.25511]  SetSaturation=off  Saturation=[0.6404,0.7127,0.8441,0.9214,0.9956,1.082,1.19,1.316,1.457;0.7,0.7698,0.8872,0.9466,0.9969,1.046,1.1,1.151,1.201]  LoadFlowParameters=[2 4000000000 0 0 0]  TsPowergui=0  TsBlock=-1  IterativeModel=Trapezoidal non iterative  IterativeDiscreteModel=Trapezoidal non iterative  BusType=swing  Pref=0  Qref=0  Qmin=-Inf  Qmax=Inf  PLF=0  QLF=0
      settings: AttributesFormatString=\n\n
  LG3 660 Mvar : powerlib/Elements/Three-Phase Series RLC Load  LConnTagsString=A|B|C  Configuration=Y (grounded)  NominalVoltage=735e3  Vabc=[1e3 1e3 1e3]  Vabcp=[1e3 1e3 1e3]  NominalFrequency=60  UnbalancedPower=off  ActivePower=2200000  InductivePower=660e6  CapacitivePower=0  Pabc=[10e3 9e3 11e3]  QLabc=[100 90 110]  QCabc=[100 90 110]  Pabcp=[10e3 9e3 11e3]  QLabcp=[100 90 110]  QCabcp=[100 90 110]  Measurements=None  LoadType=constant Z
  LG3-LMO 104km : powerlib/Elements/Distributed Parameters Line  Phases=3  Length=104  Frequency=60  Resistance="[0.01273  0.3864]"  Inductance="[0.9337e-3  4.1264e-3]"  Capacitance=[12.74e-9 7.751e-9]  x1=[-0.0006 2.03624292282842e-09 0 0;-0.00056 1.93781290190637e-09 0 0;-0.00052 1.83894223904141e-09 0 0;-0.00048 1.73965341656965e-09 0 0;-0.00044 1.6399690119131e-09 0 0;-0.0004 1.53991169244573e-09 0 0;-0.00036 1.43950421033913e-09 550361.292729253 -486648.874020806;-0.00032 1.33876939738886e-09 557636.96604399 -478294.603154611;-0.00028 1.23773015982267e-09 564785.837521505 -469831.572220297;-0.00024 1.13640947309187e-09 571806.281570074 -461261.705638114;-0.0002 1.03483037664687e-09 578696.701801261 -452586.952121821;-0.00016 9.33015968698214e-10 585455.531392926 -443809.284235559;-0.00012 8.30989400964265e-10 592081.233445506 -434930.69794531;-8e-05 7.28773873406683e-10 598572.301331491 -425953.21216503;-4e-05 6.26392628954967e-10 604927.259038022 -416878.868297569]  x2=[-0.0006 2.86206431652288e-08 0 0;-0.00056 2.85717019502185e-08 0 0;-0.00052 2.85162637765766e-08 0 0;-0.00048 2.84543412504657e-08 0 0;-0.00044 2.83859484525342e-08 0 0;-0.0004 2.83111009347146e-08 0 0;-0.00036 2.8229815716687e-08 509416.858097929 -556033.052303048;-0.00032 2.81421112820089e-08 517743.436836718 -548288.300412632;-0.00028 2.80480075739126e-08 525952.2851828 -540418.87249094;-0.00024 2.79475259907697e-08 534041.536514851 -532426.557978017;-0.0002 2.78406893812256e-08 542009.351406876 -524313.17425726;-0.00016 2.77275220390042e-08 549853.918046481 -516080.566242162;-0.00012 2.7608049697383e-08 557573.45264686 -507730.60595679;-8e-05 2.74822995233424e-08 565166.199852416 -499265.192110105;-4e-05 2.73503001113874e-08 572630.433137911 -490686.249664214]  x3=[-0.0006 2.16143954463044e-11 0 0;-0.00056 2.38357172848777e-11 0 0;-0.00052 2.60516190868908e-11 0 0;-0.00048 2.82615969753832e-11 0 0;-0.00044 3.0465148420441e-11 0 0;-0.0004 3.26617723534683e-11 0 0;-0.00036 3.48509692811255e-11 -30.2154771365785 -878.894027386153;-0.00032 3.70322413989102e-11 -16.9589161282642 -879.249677065184;-0.00028 3.92050927043532e-11 -3.6984988086698 -879.405392949977;-0.00024 4.13690291098055e-11 9.56275951765919 -879.361139632082;-0.0002 4.35235585547896e-11 22.8218433549396 -879.116927174322;-0.00016 4.56681911178895e-11 36.0757377018483 -878.672811108504;-0.00012 4.78024391281549e-11 49.3214287371075 -878.028892422791;-8e-05 4.99258172759933e-11 62.5559045048017 -877.185317538741;-4e-05 5.20378427235249e-11 75.7761555992707 -876.142278278006]  x4=[-0.0006 1.84249790225642e-11 0 0;-0.00056 1.60704418965893e-11 0 0;-0.00052 1.37122504907128e-11 0 0;-0.00048 1.13509410373241e-11 0 0;-0.00044 8.98705047782989e-12 0 0;-0.0004 6.62111634055802e-12 0 0;-0.00036 4.25367661852836e-12 3670.37159989683 -3222.94831504733;-0.00032 1.88526964711781e-12 3718.55339648942 -3167.23609882441;-0.00028 -4.83566018352617e-13 3765.88962610709 -3110.80368042569;-0.00024 -2.85229172508057e-12 3812.36952489943 -3053.66389209648;-0.0002 -5.22036884526736e-12 3857.98252373828 -2995.82972693187;-0.00016 -7.58725889859728e-12 3902.71825062106 -2937.3143359223;-0.00012 -9.95242367468339e-12 3946.56653302926 -2878.13102496306;-8e-05 -1.23153253554519e-11 3989.51740024158 -2818.29325182868;-4e-05 -1.46754266374375e-11 4031.56108560123 -2757.81462311277]  x5=0.000588163229675572  V1=ones(3,3)  V2=ones(3,3)  I1=ones(3,3)  I2=ones(3,3)  nHarmo=1  Measurements=None  Decoupling=off  VsMag0=0  VrMag0=0  VsAngle0=0  VrAngle0=0  IsMag0=0  IrMag0=0  IsAngle0=0  IrAngle0=0
      settings: AttributesFormatString=\n
  LG31-200 MVA : powerlib/Machines/Synchronous Machine pu Standard  PresetModel=No  MechanicalLoad=Mechanical power Pm  ShowDetailedParameters=on  RotorType=Salient-pole  Units=per unit standard parameters  MeasurementBus=off  NominalParameters="[200E6  13800   60 ]"  Reactances1=[ 31 32 33 34 35 36 37 ]  Reactances2=[ 1.305, 0.296, 0.252, 0.474, 0.243, 0.18 ]  dAxisTimeConstants=Short-circuit  qAxisTimeConstants=Open-circuit  TimeConstants1=[]  TimeConstants2=[]  TimeConstants3=[]  TimeConstants4=[]  TimeConstants5=[ 1.01, 0.053, 0.1 ]  TimeConstants6=[]  TimeConstants7=[]  TimeConstants8=[]  StatorResistance=2.8544e-3  Mechanical="[ 3.2  0  32]"  PolePairs=32  InitialConditions=[0 -65.0253 0.900243 0.900243 0.900243 0.798134 -119.202 120.798 1.40505]  SetSaturation=off  Saturation=[0.6404,0.7127,0.8441,0.9214,0.9956,1.082,1.19,1.316,1.457;0.7,0.7698,0.8872,0.9466,0.9969,1.046,1.1,1.151,1.201]  LoadFlowParameters=[1 180000000 0 0 0]  TsPowergui=0  TsBlock=-1  IterativeModel=Trapezoidal non iterative  IterativeDiscreteModel=Trapezoidal non iterative  BusType=PV  Pref=180000000  Qref=0  Qmin=-Inf  Qmax=Inf  PLF=0  QLF=0
      settings: AttributesFormatString=\n\n
  LG3_2200 MVA : powerlib/Machines/Synchronous Machine pu Standard  PresetModel=No  MechanicalLoad=Mechanical power Pm  ShowDetailedParameters=on  RotorType=Salient-pole  Units=per unit standard parameters  MeasurementBus=off  NominalParameters="[2200E6  13800   60 ]"  Reactances1=[ 31 32 33 34 35 36 37 ]  Reactances2=[ 1.305, 0.296, 0.252, 0.474, 0.243, 0.18 ]  dAxisTimeConstants=Short-circuit  qAxisTimeConstants=Open-circuit  TimeConstants1=[]  TimeConstants2=[]  TimeConstants3=[]  TimeConstants4=[]  TimeConstants5=[ 1.01, 0.053, 0.1 ]  TimeConstants6=[]  TimeConstants7=[]  TimeConstants8=[]  StatorResistance=2.8544e-3  Mechanical="[ 3.2  0  32]"  PolePairs=32  InitialConditions=[0 -67.4267 0.818333 0.818333 0.818333 0.465769 -119.534 120.466 1.33761]  SetSaturation=off  Saturation=[0.6404,0.7127,0.8441,0.9214,0.9956,1.082,1.19,1.316,1.457;0.7,0.7698,0.8872,0.9466,0.9969,1.046,1.1,1.151,1.201]  LoadFlowParameters=[1 1800000000 0 0 0]  TsPowergui=0  TsBlock=-1  IterativeModel=Trapezoidal non iterative  IterativeDiscreteModel=Trapezoidal non iterative  BusType=PV  Pref=1800000000  Qref=0  Qmin=-Inf  Qmax=Inf  PLF=0  QLF=0
      settings: AttributesFormatString=\n\n
  LG4 660 Mvar : powerlib/Elements/Three-Phase Series RLC Load  LConnTagsString=A|B|C  Configuration=Y (grounded)  NominalVoltage=735e3  Vabc=[1e3 1e3 1e3]  Vabcp=[1e3 1e3 1e3]  NominalFrequency=60  UnbalancedPower=off  ActivePower=2200000  InductivePower=660e6  CapacitivePower=0  Pabc=[10e3 9e3 11e3]  QLabc=[100 90 110]  QCabc=[100 90 110]  Pabcp=[10e3 9e3 11e3]  QLabcp=[100 90 110]  QCabcp=[100 90 110]  Measurements=None  LoadType=constant Z
  LG4-2700 MVA : powerlib/Machines/Synchronous Machine pu Standard  PresetModel=No  MechanicalLoad=Mechanical power Pm  ShowDetailedParameters=on  RotorType=Salient-pole  Units=per unit standard parameters  MeasurementBus=off  NominalParameters="[2700E6  13800   60 ]"  Reactances1=[ 31 32 33 34 35 36 37 ]  Reactances2=[ 1.305, 0.296, 0.252, 0.474, 0.243, 0.18 ]  dAxisTimeConstants=Short-circuit  qAxisTimeConstants=Open-circuit  TimeConstants1=[]  TimeConstants2=[]  TimeConstants3=[]  TimeConstants4=[]  TimeConstants5=[ 1.01, 0.053, 0.1 ]  TimeConstants6=[]  TimeConstants7=[]  TimeConstants8=[]  StatorResistance=2.8544e-3  Mechanical="[ 3.7  0  32]"  PolePairs=32  InitialConditions=[0 -66.0751 0.928325 0.928325 0.928325 3.71347 -116.287 123.713 1.33221]  SetSaturation=off  Saturation=[0.6404,0.7127,0.8441,0.9214,0.9956,1.082,1.19,1.316,1.457;0.7,0.7698,0.8872,0.9466,0.9969,1.046,1.1,1.151,1.201]  LoadFlowParameters=[1 2500000000 0 0 0]  TsPowergui=0  TsBlock=-1  IterativeModel=Trapezoidal non iterative  IterativeDiscreteModel=Trapezoidal non iterative  BusType=PV  Pref=2500000000  Qref=0  Qmin=-Inf  Qmax=Inf  PLF=0  QLF=0
      settings: AttributesFormatString=\n\n
  LG4-LMO 3*118km : powerlib/Elements/Distributed Parameters Line  Phases=3  Length=118  Frequency=60  Resistance="[0.01273  0.3864]/3"  Inductance="[0.9337e-3  4.1264e-3]/3"  Capacitance=[12.74e-9 7.751e-9]*3  x1=[-0.00068 3.57284971337298e-09 0 0;-0.00064 3.564221369762e-09 0 0;-0.0006 3.55478255294807e-09 0 0;-0.00056 3.54453540923674e-09 0 0;-0.00052 3.53348226874013e-09 0 0;-0.00048 3.52162564484705e-09 0 0;-0.00044 3.50896823365154e-09 516886.507538865 -533088.832052363;-0.0004 3.49551291333976e-09 524866.260233761 -525234.058896104;-0.00036 3.4812627435355e-09 532726.662867333 -517259.852044277;-0.00032 3.46622096460449e-09 540465.928051808 -509168.024762754;-0.00028 3.45039099691754e-09 548082.295945024 -500960.417063278;-0.00024 3.43377644007281e-09 555574.034650602 -492638.895285061;-0.0002 3.41638107207722e-09 562939.440611768 -484205.351670393;-0.00016 3.39820884848746e-09 570176.838998721 -475661.703934364;-0.00012 3.37926390151046e-09 577284.584089481 -467009.894828792;-8e-05 3.35955053906379e-09 584261.05964411 -458251.891700458;-4e-05 3.33907324379607e-09 591104.679272229 -449389.686043747]  x2=[-0.00068 2.86722039265522e-08 0 0;-0.00064 2.86343709619278e-08 0 0;-0.0006 2.85900267882789e-08 0 0;-0.00056 2.85391814890883e-08 0 0;-0.00052 2.84818466261385e-08 0 0;-0.00048 2.84180352368829e-08 0 0;-0.00044 2.83477618314811e-08 492418.109351363 -571141.512381592;-0.0004 2.82710423894995e-08 500974.442358633 -563651.367072395;-0.00036 2.81878943562776e-08 509416.858097929 -556033.052303048;-0.00032 2.80983366389612e-08 517743.436836719 -548288.300412632;-0.00028 2.80023896022028e-08 525952.2851828 -540418.87249094;-0.00024 2.79000750635312e-08 534041.536514851 -532426.557978017;-0.0002 2.77914162883901e-08 542009.351406876 -524313.17425726;-0.00016 2.76764379848481e-08 549853.918046481 -516080.566242162;-0.00012 2.75551662979797e-08 557573.45264686 -507730.60595679;-8e-05 2.74276288039208e-08 565166.199852416 -499265.192110105;-4e-05 2.72938545035976e-08 572630.433137912 -490686.249664214]  x3=[-0.00068 1.31979718323151e-10 0 0;-0.00064 1.37556975464631e-10 0 0;-0.0006 1.4310295333613e-10 0 0;-0.00056 1.48616390830109e-10 0 0;-0.00052 1.54096034238425e-10 0 0;-0.00048 1.59540637537424e-10 0 0;-0.00044 1.64948962671266e-10 2439.66221449294 -4653.85507160121;-0.0004 1.70319779833457e-10 2509.56057642216 -4616.53818277179;-0.00036 1.75651867746488e-10 2578.88828591782 -4578.17153297094;-0.00032 1.80944013939551e-10 2647.62957845666 -4538.76384644397;-0.00028 1.86195015024239e-10 2715.76882286153 -4498.32408415894;-0.00024 1.91403676968188e-10 2783.29052485588 -4456.86144176907;-0.0002 1.96568815366589e-10 2850.17933058696 -4414.38534752168;-0.00016 2.01689255711513e-10 2916.42003011715 -4370.90546011431;-0.00012 2.06763833658982e-10 2981.99756088264 -4326.43166649838;-8e-05 2.11791395293733e-10 3046.89701111843 -4280.97407963105;-4e-05 2.16770797391605e-10 3111.10362324921 -4234.54303617556]  x4=[-0.00068 -1.20540634814595e-12 0 0;-0.00064 -6.69288500676156e-12 0 0;-0.0006 -1.21788417610436e-11 0 0;-0.00056 -1.7662029151735e-11 0 0;-0.00052 -2.31412003493082e-11 0 0;-0.00048 -2.86151094374831e-11 0 0;-0.00044 -3.40825116965382e-11 7760.55546914452 -8389.19553241511;-0.0004 -3.95421638863486e-11 7886.17526884407 -8271.21966070313;-0.00036 -4.49928245290882e-11 8010.00182029496 -8151.36298496826;-0.00032 -5.04332541915316e-11 8132.00696640723 -8029.65275958497;-0.00028 -5.58622157668897e-11 8252.16296426278 -7906.11666040893;-0.00024 -6.12784747561176e-11 8370.44249142389 -7780.78277848376;-0.0002 -6.6680799548629e-11 8486.81865214606 -7653.67961365337;-0.00016 -7.20679617023538e-11 8601.26498349394 -7524.83606808136;-0.00012 -7.74387362230751e-11 8713.75546135873 -7394.2814396789;-8e-05 -8.27919018429825e-11 8824.26450637582 -7262.04541544261;-4e-05 -8.81262412983778e-11 8932.76698974139 -7128.15806470407]  x5=0.000667339049054976  V1=ones(3,3)  V2=ones(3,3)  I1=ones(3,3)  I2=ones(3,3)  nHarmo=1  Measurements=None  Decoupling=off  VsMag0=0  VrMag0=0  VsAngle0=0  VrAngle0=0  IsMag0=0  IrMag0=0  IsAngle0=0  IrAngle0=0
      settings: AttributesFormatString=\n
  LMO 330 Mvar : powerlib/Elements/Three-Phase Series RLC Load  LConnTagsString=A|B|C  Configuration=Y (grounded)  NominalVoltage=735e3  Vabc=[1e3 1e3 1e3]  Vabcp=[1e3 1e3 1e3]  NominalFrequency=60  UnbalancedPower=off  ActivePower=1100000  InductivePower=330e6  CapacitivePower=0  Pabc=[10e3 9e3 11e3]  QLabc=[100 90 110]  QCabc=[100 90 110]  Pabcp=[10e3 9e3 11e3]  QLabcp=[100 90 110]  QCabcp=[100 90 110]  Measurements=None  LoadType=constant Z
  LMO-ALB 3*218km : powerlib/Elements/Distributed Parameters Line  Phases=3  Length=218  Frequency=60  Resistance="[0.01273  0.3864]/3"  Inductance="[0.9337e-3  4.1264e-3]/3"  Capacitance=[12.74e-9 7.751e-9]*3  x1=[-0.00124 2.84830372626674e-08 300539.143349299 -691631.439095048;-0.0012 2.85385532753212e-08 310934.166982576 -687020.941454766;-0.00116 2.85875798670662e-08 321258.486867662 -682254.221177013;-0.00112 2.86301058896782e-08 331509.75534325 -677332.362172875;-0.00108 2.86661216731064e-08 341685.641359291 -672256.483630643;-0.00104 2.86956190276723e-08 351783.831007058 -667027.739761328;-0.001 2.87185912459318e-08 361802.028045309 -661647.319536192;-0.00096 2.87350331042005e-08 371737.954422431 -656116.446416398;-0.00092 2.87449408637417e-08 381589.350794448 -650436.378074796;-0.00088 2.87483122716163e-08 391353.977038781 -644608.406109944;-0.00084 2.87451465611952e-08 401029.612763628 -638633.855752408;-0.0008 2.87354444523336e-08 410614.057812865 -632514.085563419;-0.00076 2.87192081512076e-08 420105.132766341 -626250.487125941;-0.00072 2.86964413498118e-08 429500.679435457 -619844.484728246;-0.00068 2.86671492251207e-08 438798.561353926 -613297.535040034;-0.00064 2.86313384379108e-08 447996.664263581 -606611.126781207;-0.0006 2.85890171312462e-08 457092.896595141 -599786.780383341;-0.00056 2.85401949286271e-08 466085.189943816 -592826.047643957;-0.00052 2.84848829318015e-08 474971.499539646 -585730.511373653;-0.00048 2.84230937182403e-08 483749.80471246 -578501.785036188;-0.00044 2.83548413382779e-08 492418.109351363 -571141.512381592;-0.0004 2.8280141311917e-08 500974.442358632 -563651.367072395;-0.00036 2.81990106252992e-08 509416.858097929 -556033.052303048;-0.00032 2.81114677268432e-08 517743.436836718 -548288.300412632;-0.00028 2.8017532523049e-08 525952.2851828 -540418.87249094;-0.00024 2.79172263739721e-08 534041.536514851 -532426.557978017;-0.0002 2.78105720883656e-08 542009.351406876 -524313.17425726;-0.00016 2.76975939184943e-08 549853.918046481 -516080.566242162;-0.00012 2.75783175546199e-08 557573.45264686 -507730.60595679;-8e-05 2.74527701191588e-08 565166.199852416 -499265.192110105;-4e-05 2.73209801605152e-08 572630.433137911 -490686.249664214]  x2=[-0.00124 8.85352618407578e-08 180359.157644513 -744264.312744397;-0.0012 8.87728810437979e-08 191561.495110343 -741460.025520597;-0.00116 8.89903140592332e-08 202720.273144142 -738487.136681071;-0.00112 8.91875114446714e-08 213832.954336013 -735346.322235106;-0.00108 8.93644283591273e-08 224897.011758084 -732038.296376822;-0.00104 8.95210245732204e-08 235909.929539111 -728563.811322771;-0.001 8.9657264478322e-08 246869.203436562 -724923.657140892;-0.00096 8.97731170946525e-08 257772.34140606 -721118.661570854;-0.00092 8.98685560783261e-08 268616.864168057 -717149.689835838;-0.00088 8.99435597273408e-08 279400.305771595 -713017.644445788;-0.00084 8.99981109865139e-08 290120.214155046 -708723.464992194;-0.0008 9.00321974513592e-08 300774.151703688 -704268.127934432;-0.00076 9.00458113709087e-08 311359.695803999 -699652.646377726;-0.00072 9.00389496494745e-08 321874.439394535 -694878.069842782;-0.00068 9.00116138473528e-08 332315.991513281 -689945.484027129;-0.00064 8.99638101804693e-08 342681.977841327 -684856.010558245;-0.0006 8.98955495189656e-08 352970.041242775 -679610.806738506;-0.00056 8.98068473847276e-08 363177.842300729 -674211.065282029;-0.00052 8.96977239478555e-08 373303.059849257 -668658.014043456;-0.00048 8.95682040220779e-08 383343.391501202 -662952.91573875;-0.00044 8.94183170591089e-08 393296.554171733 -657097.067658068;-0.0004 8.92480971419515e-08 403160.284597491 -651091.801370764;-0.00036 8.90575829771467e-08 412932.339851237 -644938.482422604;-0.00032 8.88468178859729e-08 422610.497851878 -638638.510025255;-0.00028 8.86158497945941e-08 432192.557869745 -632193.31673811;-0.00024 8.83647312231626e-08 441676.341027023 -625604.368142541;-0.0002 8.80935192738759e-08 451059.690793205 -618873.162508639;-0.00016 8.78022756179925e-08 460340.473475474 -612001.230454518;-0.00012 8.74910664818081e-08 469516.578703882 -604990.134598265;-8e-05 8.71599626315966e-08 478585.919911232 -597841.469202617;-4e-05 8.68090393575182e-08 487546.434807542 -590556.859812438]  x3=[-0.00124 1.17950397412832e-10 -23.6154950525097 -3420.19245713402;-0.0012 1.26306249080514e-10 27.9605314484087 -3420.15971859338;-0.00116 1.34633379796374e-10 79.530199965597 -3419.34926522694;-0.00112 1.42929896042696e-10 131.081784001153 -3417.7612813248;-0.00108 1.51193911263233e-10 182.603561169427 -3415.39612798081;-0.00104 1.5942354629219e-10 234.083815862598 -3412.25434301044;-0.001 1.6761692978153e-10 285.510841914694 -3408.33664082849;-0.00096 1.75772198626505e-10 336.87294526348 -3403.64391228666;-0.00092 1.83887498389307e-10 388.158446609581 -3398.17722447095;-0.00088 1.91960983720753e-10 439.35568407226 -3391.93782045903;-0.00084 1.99990818779903e-10 490.453015841222 -3384.92711903756;-0.0008 2.07975177651509e-10 541.438822823868 -3377.1467143796;-0.00076 2.15912244761219e-10 592.301511287374 -3368.59837568205;-0.00072 2.23800215288418e-10 643.029515495004 -3359.28404676343;-0.00068 2.31637295576631e-10 693.611300336061 -3349.20584562181;-0.00064 2.39421703541385e-10 744.03536394887 -3338.36606395322;-0.0006 2.47151669075438e-10 794.290240336205 -3326.76716663052;-0.00056 2.54825434451289e-10 844.364501972556 -3314.41179114295;-0.00052 2.62441254720867e-10 894.246762402646 -3301.30274699635;-0.00048 2.69997398112318e-10 943.925678830623 -3287.4430150743;-0.00044 2.77492146423797e-10 993.389954699301 -3272.83574696032;-0.0004 2.8492379541417e-10 1042.62834225891 -3257.48426422122;-0.00036 2.92290655190543e-10 1091.62964512473 -3241.39205765178;-0.00032 2.99591050592533e-10 1140.38272082307 -3224.56278648101;-0.00028 3.06823321573182e-10 1188.87648332493 -3207.00027754004;-0.00024 3.13985823576437e-10 1237.09990556692 -3188.70852439194;-0.0002 3.21076927911109e-10 1285.04202195868 -3169.69168642365;-0.00016 3.28095022121223e-10 1332.69193087637 -3149.95408790013;-0.00012 3.35038510352678e-10 1380.03879714163 -3129.50021698106;-8e-05 3.41905813716128e-10 1427.07185448537 -3108.33472470031;-4e-05 3.48695370646009e-10 1473.78040799594 -3086.46242390831]  x4=[-0.00124 3.05311377390038e-10 3052.91388647781 -13125.664701462;-0.0012 2.99603497299669e-10 3250.49024737001 -13078.1368217818;-0.00116 2.93827489957683e-10 3447.327474811 -13027.6350865694;-0.00112 2.87984668778342e-10 3643.38080971271 -12974.1709794838;-0.00108 2.82076362368795e-10 3838.60567123746 -12917.756657802;-0.00104 2.76103914226968e-10 4032.9576669353 -12858.4049496542;-0.001 2.70068682436065e-10 4226.39260283842 -12796.129351107;-0.00096 2.63972039355748e-10 4418.86649351052 -12730.9440230945;-0.00092 2.57815371310081e-10 4610.33557204867 -12662.8637881982;-0.00088 2.51600078272282e-10 4800.75630003558 -12591.9041272762;-0.00084 2.45327573546391e-10 4990.08537743982 -12518.0811759437;-0.0008 2.3899928344589e-10 5178.27975246189 -12441.4117209031;-0.00076 2.32616646969376e-10 5365.29663132384 -12361.9131961274;-0.00072 2.26181115473341e-10 5551.09348800017 -12279.6036788954;-0.00068 2.19694152342151e-10 5735.62807388792 -12194.5018856817;-0.00064 2.1315723265528e-10 5918.85842741362 -12106.6271679;-0.0006 2.06571842851892e-10 6100.74288357499 -12015.9995075035;-0.00056 1.9993948039284e-10 6281.2400834152 -11922.6395124405;-0.00052 1.93261653420151e-10 6460.30898342754 -11826.5684119689;-0.00048 1.86539880414092e-10 6637.90886488839 -11727.8080518284;-0.00044 1.79775689847878e-10 6813.99934311625 -11626.3808892732;-0.0004 1.72970619840112e-10 6988.54037665491 -11522.3099879654;-0.00036 1.6612621780503e-10 7161.49227637853 -11415.6190127305;-0.00032 1.5924404010063e-10 7332.81571451658 -11306.3322241763;-0.00028 1.52325651674774e-10 7502.47173359665 -11194.4744731759;-0.00024 1.45372625709327e-10 7670.42175530307 -11080.0711952173;-0.0002 1.38386543262434e-10 7836.62758924923 -10963.1484046194;-0.00016 1.31368992908998e-10 8001.05144166179 -10843.7326886165;-0.00012 1.24321570379452e-10 8163.65592397465 -10721.8512013126;-8e-05 1.17245878196906e-10 8324.40406133077 -10597.5316575067;-4e-05 1.10143525312743e-10 8483.25930098994 -10470.8023263912]  x5=0.00123288061605072  V1=ones(3,3)  V2=ones(3,3)  I1=ones(3,3)  I2=ones(3,3)  nHarmo=1  Measurements=None  Decoupling=off  VsMag0=0  VrMag0=0  VsAngle0=0  VrAngle0=0  IsMag0=0  IrMag0=0  IsAngle0=0  IrAngle0=0
      settings: AttributesFormatString=\n
  LMO7 : powerlib/Measurements/Three-Phase V-I Measurement  VoltageMeasurement=no  SetLabelV=on  LabelV=Vabc_LMO7  Vpu=on  VpuLL=off  CurrentMeasurement=no  SetLabelI=off  LabelI=A1  Ipu=off  Pbase=100e6  Vbase=735e3  OutputType=Magnitude  PhasorSimulation=off  PSBequivalent=0
  LVD 990 Mvar : powerlib/Elements/Three-Phase Series RLC Load  LConnTagsString=A|B|C  Configuration=Y (grounded)  NominalVoltage=735e3  Vabc=[1e3 1e3 1e3]  Vabcp=[1e3 1e3 1e3]  NominalFrequency=60  UnbalancedPower=off  ActivePower=3300000  InductivePower=990e6  CapacitivePower=0  Pabc=[10e3 9e3 11e3]  QLabc=[100 90 110]  QCabc=[100 90 110]  Pabcp=[10e3 9e3 11e3]  QLabcp=[100 90 110]  QCabcp=[100 90 110]  Measurements=None  LoadType=constant Z
  LVD-MTL 3*260km : powerlib/Elements/Distributed Parameters Line  Phases=3  Length=260  Frequency=60  Resistance="[0.01273  0.3864]/3"  Inductance="[0.9337e-3  4.1264e-3]/3"  Capacitance=[12.74e-9 7.751e-9]*3  x1=[-0.00148 2.75789889916239e-07 -29973.8950598746 -777968.644211563;-0.00144 2.77115476270194e-07 -18239.4210694087 -778332.145881461;-0.0014 2.78378048954586e-07 -6500.79959188168 -778518.661533437;-0.00136 2.79577320871277e-07 5239.30011141196 -778528.148755439;-0.00132 2.80713019316173e-07 16978.2084430421 -778360.605390154;-0.00128 2.81784886041243e-07 28713.2560764862 -778016.0695355;-0.00124 2.82792677313237e-07 40441.774563111 -777494.619535959;-0.0012 2.83736163969109e-07 52161.0969389552 -776796.373964763;-0.00116 2.84615131468132e-07 63868.5583311736 -775921.491596934;-0.00112 2.85429379940675e-07 75561.4965640064 -774870.171373178;-0.00108 2.86178724233657e-07 87237.2527641352 -773642.652354647;-0.00104 2.86862993952649e-07 98893.1719652875 -772239.213668581;-0.001 2.87482033500618e-07 110526.603711953 -770660.174444834;-0.00096 2.88035702113308e-07 122134.902662076 -768905.893743309;-0.00092 2.88523873891251e-07 133715.429188579 -766976.770472309;-0.00088 2.88946437828395e-07 145265.549979598 -764873.243297829;-0.00084 2.89303297837346e-07 156782.638637269 -762595.790543809;-0.0008 2.89594372771213e-07 168264.076274949 -760144.930083365;-0.00076 2.89819596442068e-07 179707.252112732 -757521.219221031;-0.00072 2.89978917635989e-07 191109.564071113 -754725.254566031;-0.00068 2.90072300124712e-07 202468.419362684 -751757.671896616;-0.00064 2.90099722673863e-07 213781.235081705 -748619.146015494;-0.0006 2.90061179047792e-07 225045.438791439 -745310.390596385;-0.00056 2.89956678010986e-07 236258.469109101 -741832.158021737;-0.00052 2.89786243326081e-07 247417.776288294 -738185.239211643;-0.00048 2.89549913748454e-07 258520.822798799 -734370.46344399;-0.00044 2.89247743017412e-07 269565.083903588 -730388.698165892;-0.0004 2.88879799843974e-07 280548.048232928 -726240.848796434;-0.00036 2.88446167895245e-07 291467.218355443 -721927.858520795;-0.00032 2.8794694577539e-07 302320.11134601 -717450.708075768;-0.00028 2.87382247003215e-07 313104.259350355 -712810.415526757;-0.00024 2.8675219998635e-07 323817.21014622 -708008.03603627;-0.0002 2.86056947992054e-07 334456.527700978 -703044.661623989;-0.00016 2.85296649114635e-07 345019.792725567 -697921.420918455;-0.00012 2.84471476239501e-07 355504.603224614 -692639.478900421;-8e-05 2.83581617003847e-07 365908.575042629 -687200.036637954;-4e-05 2.8262727375399e-07 376229.342406141 -681604.331013316]  x2=[-0.00148 4.16707701978354e-07 -239041.030981867 -695044.447394561;-0.00144 4.18543125930133e-07 -228533.218022587 -698569.915440727;-0.0014 4.20283376784437e-07 -217973.438580316 -701936.534712332;-0.00136 4.2192805882323e-07 -207364.093857835 -705143.539669186;-0.00132 4.2347679806e-07 -196707.596328642 -708190.201066018;-0.00128 4.24929242324798e-07 -186006.369188378 -711075.8261183;-0.00124 4.26285061344326e-07 -175262.845803811 -713799.75865978;-0.0012 4.2754394681703e-07 -164479.46915951 -716361.379291687;-0.00116 4.2870561248321e-07 -153658.691302334 -718760.10552358;-0.00112 4.29769794190111e-07 -142802.972783851 -720995.391905801;-0.00108 4.30736249951989e-07 -131914.782100838 -723066.730153502;-0.00104 4.3160476000514e-07 -120996.59513396 -724973.649262228;-0.001 4.32375126857867e-07 -110050.894584778 -726715.715615018;-0.00096 4.33047175335391e-07 -99080.1694112061 -728292.533081006;-0.00092 4.33620752619683e-07 -88086.9142615413 -729703.7431055;-0.00088 4.34095728284215e-07 -77073.6289072025 -730949.024791508;-0.00084 4.34471994323618e-07 -66042.8176743049 -732028.094972715;-0.0008 4.34749465178238e-07 -54996.9888741972 -732940.708277866;-0.00076 4.34928077753597e-07 -43938.6542330933 -733686.657186566;-0.00072 4.35007791434734e-07 -32870.3283209277 -734265.772076466;-0.00068 4.34988588095447e-07 -21794.5279795635 -734677.921261835;-0.00064 4.34870472102408e-07 -10713.7717504847 -734923.011023501;-0.0006 4.34653470314177e-07 369.420697898489 -735000.985630166;-0.00056 4.34337632075088e-07 11452.5291432007 -734911.827351078;-0.00052 4.33923029204034e-07 22533.0333821382 -734655.55646006;-0.00048 4.33409755978131e-07 33608.4138036012 -734232.231230902;-0.00044 4.32797929111285e-07 44676.1519615918 -733641.947924112;-0.0004 4.3208768772765e-07 55733.7311478971 -732884.840765022;-0.00036 4.31279193329991e-07 66778.6369643666 -731961.081913272;-0.00032 4.30372629762963e-07 77808.3578946649 -730870.881423659;-0.00028 4.29368203171301e-07 88820.3858753686 -729614.487198372;-0.00024 4.28266141952953e-07 99812.2168662786 -728192.184930623;-0.0002 4.27066696707133e-07 110781.351419817 -726604.298039683;-0.00016 4.2577014017735e-07 121725.29524938 -724851.187597338;-0.00012 4.24376767189375e-07 132641.559796518 -722933.252245783;-8e-05 4.2288689458421e-07 143527.662796811 -720850.928106978;-4e-05 4.21300861146039e-07 154381.128844313 -718604.688683476]  x3=[-0.00148 9.07372967752802e-10 714.210166669584 -1454.18503773149;-0.00144 9.32309877055665e-10 736.056871921486 -1443.25012675928;-0.0014 9.57034787132384e-10 757.736204188198 -1431.9870331543;-0.00136 9.81542075751625e-10 779.243233776515 -1420.39831804691;-0.00132 1.0058261701673e-09 800.57307017338 -1408.486616611;-0.00128 1.02988154838575e-09 821.720863157935 -1396.25463746473;-0.00124 1.05370274042142e-09 842.681803904426 -1383.7051620547;-0.0012 1.07728432954067e-09 863.451126075689 -1370.84104402338;-0.00116 1.10062095349348e-09 884.024106906967 -1357.66520856028;-0.00112 1.12370730573281e-09 904.396068279833 -1344.18065173675;-0.00108 1.14653813662127e-09 924.562377785952 -1330.39043982475;-0.00104 1.16910825462478e-09 944.518449780449 -1316.29770859952;-0.001 1.19141252749314e-09 964.259746424647 -1301.90566262663;-0.00096 1.21344588342706e-09 983.781778717929 -1287.21757453321;-0.00092 1.2352033122314e-09 1003.0801075185 -1272.23678426384;-0.00088 1.25667986645448e-09 1022.15034455282 -1256.96669832102;-0.00084 1.27787066251307e-09 1040.98815341344 -1241.41078899063;-0.0008 1.2987708818029e-09 1059.58925054507 -1225.57259355229;-0.00076 1.31937577179432e-09 1077.94940621864 -1209.45571347507;-0.00072 1.33968064711305e-09 1096.06444549307 -1193.0638135985;-0.00068 1.35968089060554e-09 1113.93024916465 -1176.40062129927;-0.00064 1.3793719543889e-09 1131.5427547037 -1159.4699256436;-0.0006 1.39874936088502e-09 1148.89795717833 -1142.27557652568;-0.00056 1.41780870383878e-09 1165.99191016518 -1124.82148379222;-0.00052 1.43654564931995e-09 1182.82072664675 -1107.1116163534;-0.00048 1.45495593670871e-09 1199.38057989528 -1089.15000128034;-0.00044 1.47303537966446e-09 1215.66770434297 -1070.94072288942;-0.0004 1.4907798670778e-09 1231.67839643816 -1052.48792181351;-0.00036 1.5081853640053e-09 1247.40901548754 -1033.79579406045;-0.00032 1.52524791258706e-09 1262.85598448399 -1014.8685900589;-0.00028 1.54196363294667e-09 1278.01579091999 -995.710613691827;-0.00024 1.55832872407349e-09 1292.88498758626 -976.32622131784;-0.0002 1.5743394646869e-09 1307.46019335572 -956.719820780603;-0.00016 1.58999221408257e-09 1321.73809395227 -936.895870406522;-0.00012 1.60528341296026e-09 1335.71544270444 -916.858877990956;-8e-05 1.62020958423322e-09 1349.38906128366 -896.613399773189;-4e-05 1.63476733381882e-09 1362.75584042698 -876.164039400378]  x4=[-0.00148 1.41913783038523e-09 -6436.59844910999 -14213.1446245357;-0.00144 1.41730566272213e-09 -6221.54551111483 -14308.5859275335;-0.0014 1.41515121197365e-09 -6005.07784732277 -14400.7735814833;-0.00136 1.41267496804331e-09 -5787.24468061381 -14489.6866237077;-0.00132 1.40987749400763e-09 -5568.09554437155 -14575.3048361476;-0.00128 1.40675942598808e-09 -5347.68027121971 -14657.6087499599;-0.00124 1.40332147300644e-09 -5126.04898169062 -14736.5796499442;-0.0012 1.39956441682356e-09 -4903.25207282827 -14812.199578799;-0.00116 1.39548911176162e-09 -4679.34020672839 -14884.4513412046;-0.00112 1.39109648450986e-09 -4454.36429901842 -14953.3185077332;-0.00108 1.38638753391383e-09 -4228.37550727966 -15018.785418585;-0.00104 1.38136333074828e-09 -4001.42521941449 -15080.8371871492;-0.001 1.37602501747368e-09 -3773.56504196125 -15139.4597033886;-0.00096 1.37037380797645e-09 -3544.84678835931 -15194.6396370486;-0.00092 1.36441098729289e-09 -3315.32246716716 -15246.3644406882;-0.00088 1.35813791131699e-09 -3085.04427023609 -15294.6223525329;-0.00084 1.35155600649214e-09 -2854.06456084226 -15339.4023991499;-0.0008 1.34466676948674e-09 -2622.4358617797 -15380.6943979427;-0.00076 1.33747176685387e-09 -2390.21084341709 -15418.4889594669;-0.00072 1.32997263467509e-09 -2157.44231172099 -15452.7774895651;-0.00068 1.32217107818837e-09 -1924.1831962482 -15483.5521913212;-0.00064 1.31406887140039e-09 -1690.48653811002 -15510.8060668335;-0.0006 1.3056678566831e-09 -1456.40547791122 -15534.5329188057;-0.00056 1.2969699443548e-09 -1221.99324366625 -15554.7273519563;-0.00052 1.28797711224575e-09 -987.303138695682 -15571.3847742452;-0.00048 1.27869140524842e-09 -752.388529505519 -15584.5013979184;-0.00044 1.26911493485249e-09 -517.302833652068 -15594.0742403688;-0.0004 1.25924987866477e-09 -282.099507595276 -15600.1011248145;-0.00036 1.24909847991394e-09 -46.8320345431779 -15602.5806807939;-0.00032 1.23866304694055e-09 188.446087709713 -15601.5123444774;-0.00028 1.22794595267205e-09 423.681358947348 -15596.8963587955;-0.00024 1.21694963408328e-09 658.820288697631 -15588.7337733835;-0.0002 1.20567659164224e-09 893.809408395688 -15577.026444343;-0.00016 1.19412938874157e-09 1128.59528354216 -15561.7770338196;-0.00012 1.18231065111564e-09 1363.12452585375 -15542.9890093977;-8e-05 1.17022306624345e-09 1597.34380540324 -15520.6666433121;-4e-05 1.15786938273758e-09 1831.19986274629 -15494.8150114764]  x5=0.00147040807418893  V1=ones(3,3)  V2=ones(3,3)  I1=ones(3,3)  I2=ones(3,3)  nHarmo=1  Measurements=None  Decoupling=off  VsMag0=0  VrMag0=0  VsAngle0=0  VrAngle0=0  IsMag0=0  IrMag0=0  IsAngle0=0  IrAngle0=0
      settings: AttributesFormatString=\n
  LVD7 : powerlib/Measurements/Three-Phase V-I Measurement  VoltageMeasurement=no  SetLabelV=on  LabelV=Vabc_LVD7  Vpu=on  VpuLL=off  CurrentMeasurement=no  SetLabelI=off  LabelI=A1  Ipu=off  Pbase=100e6  Vbase=735e3  OutputType=Magnitude  PhasorSimulation=off  PSBequivalent=0
  Load Flow Bus1 : powerlib/Measurements/Load Flow Bus  LConnTagsString=a  Phases=single  Connectors=on one side  ID=LG31_13.8  Vbase=13.8e3  Vref=1  Vangle=0  VLF=1  VLFb=1  VLFc=1  angleLF=2.13  angleLFb=0  angleLFc=0
      settings: AttributesFormatString=%<ID>\n%<Vbase>V\n%<VLF>pu\n%<angleLF>deg.
  Load Flow Bus10 : powerlib/Measurements/Load Flow Bus  LConnTagsString=a  Phases=single  Connectors=on one side  ID=LVD7  Vbase=735e3  Vref=1  Vangle=0  VLF=1.053  VLFb=1  VLFc=1  angleLF=-6.263  angleLFb=0  angleLFc=0
      settings: AttributesFormatString=%<ID>\n%<Vbase>V\n%<VLF>pu\n%<angleLF>deg.
  Load Flow Bus11 : powerlib/Measurements/Load Flow Bus  LConnTagsString=a  Phases=single  Connectors=on one side  ID=CHM7  Vbase=735e3  Vref=1  Vangle=0  VLF=1.055  VLFb=1  VLFc=1  angleLF=1.134  angleLFb=0  angleLFc=0
      settings: AttributesFormatString=%<ID>\n%<Vbase>V\n%<VLF>pu\n%<angleLF>deg.
  Load Flow Bus12 : powerlib/Measurements/Load Flow Bus  LConnTagsString=a  Phases=single  Connectors=on one side  ID=LG47  Vbase=735e3  Vref=1  Vangle=0  VLF=1.01  VLFb=1  VLFc=1  angleLF=23.62  angleLFb=0  angleLFc=0
      settings: AttributesFormatString=%<ID>\n%<Vbase>V\n%<VLF>pu\n%<angleLF>deg.
  Load Flow Bus2 : powerlib/Measurements/Load Flow Bus  LConnTagsString=a  Phases=single  Connectors=on one side  ID=LG3_13.8  Vbase=13.8e3  Vref=1  Vangle=0  VLF=1  VLFb=1  VLFc=1  angleLF=1.566  angleLFb=0  angleLFc=0
      settings: AttributesFormatString=%<ID>\n%<Vbase>V\n%<VLF>pu\n%<angleLF>deg.
  Load Flow Bus3 : powerlib/Measurements/Load Flow Bus  LConnTagsString=a  Phases=single  Connectors=on one side  ID=LG4_13.8  Vbase=13.8e3  Vref=1  Vangle=0  VLF=1  VLFb=1  VLFc=1  angleLF=-0.4067  angleLFb=0  angleLFc=0
      settings: AttributesFormatString=%<ID>\n%<Vbase>V\n%<VLF>pu\n%<angleLF>deg.
  Load Flow Bus4 : powerlib/Measurements/Load Flow Bus  LConnTagsString=a  Phases=single  Connectors=on one side  ID=LG2_13.8  Vbase=13.8e3  Vref=1  Vangle=0  VLF=1  VLFb=1  VLFc=1  angleLF=0  angleLFb=0  angleLFc=0
      settings: AttributesFormatString=%<ID>\n%<Vbase>V\n%<VLF>pu\n%<angleLF>deg.
  Load Flow Bus5 : powerlib/Measurements/Load Flow Bus  LConnTagsString=a  Phases=single  Connectors=on one side  ID=LG27  Vbase=735e3  Vref=1  Vangle=0  VLF=1.009  VLFb=1  VLFc=1  angleLF=24.74  angleLFb=0  angleLFc=0
      settings: AttributesFormatString=%<ID>\n%<Vbase>V\n%<VLF>pu\n%<angleLF>deg.
  Load Flow Bus6 : powerlib/Measurements/Load Flow Bus  LConnTagsString=a  Phases=single  Connectors=on one side  ID=LG37  Vbase=735e3  Vref=1  Vangle=0  VLF=0.9995  VLFb=1  VLFc=1  angleLF=26.29  angleLFb=0  angleLFc=0
      settings: AttributesFormatString=%<ID>\n%<Vbase>V\n%<VLF>pu\n%<angleLF>deg.
  Load Flow Bus7 : powerlib/Measurements/Load Flow Bus  LConnTagsString=a  Phases=single  Connectors=on one side  ID=LMO7  Vbase=735e3  Vref=1  Vangle=0  VLF=1.026  VLFb=1  VLFc=1  angleLF=20.27  angleLFb=0  angleLFc=0
      settings: AttributesFormatString=%<ID>\n%<Vbase>V\n%<VLF>pu\n%<angleLF>deg.
  Load Flow Bus8 : powerlib/Measurements/Load Flow Bus  LConnTagsString=a  Phases=single  Connectors=on one side  ID=NEM_ALB7  Vbase=735e3  Vref=1  Vangle=0  VLF=1.043  VLFb=1  VLFc=1  angleLF=12.43  angleLFb=0  angleLFc=0
      settings: AttributesFormatString=%<ID>\n%<Vbase>V\n%<VLF>pu\n%<angleLF>deg.
  Load Flow Bus9 : powerlib/Measurements/Load Flow Bus  LConnTagsString=a  Phases=single  Connectors=on one side  ID=ABI_CHB7  Vbase=735e3  Vref=1  Vangle=0  VLF=1.059  VLFb=1  VLFc=1  angleLF=4.701  angleLFb=0  angleLFc=0
      settings: AttributesFormatString=%<ID>\n%<Vbase>V\n%<VLF>pu\n%<angleLF>deg.
  NEM-ABI 6*236 : powerlib/Elements/Distributed Parameters Line  Phases=3  Length=236  Frequency=60  Resistance="[0.01273  0.3864]/6"  Inductance="[0.9337e-3  4.1264e-3]/6"  Capacitance=[12.74e-9 7.751e-9]*6  x1=[-0.00136 8.52532712138755e-08 0 0;-0.00132 8.55489825044912e-08 0 0;-0.00128 8.58252406942284e-08 0 0;-0.00124 8.60819829643571e-08 0 0;-0.0012 8.63191509338991e-08 0 0;-0.00116 8.65366906729034e-08 0 0;-0.00112 8.67345527147094e-08 0 0;-0.00108 8.69126920671949e-08 0 0;-0.00104 8.70710682230074e-08 0 0;-0.001 8.7209645168775e-08 0 0;-0.00096 8.73283913932952e-08 0 0;-0.00092 8.74272798947004e-08 0 0;-0.00088 8.75062881865984e-08 0 0;-0.00084 8.75653983031848e-08 315446.71458481 -699075.660759286;-0.0008 8.7604596803329e-08 325952.293654414 -694239.522252121;-0.00076 8.76238747736299e-08 336383.753983333 -689245.519664463;-0.00072 8.76232278304434e-08 346738.723547447 -684094.788589433;-0.00068 8.76026561208788e-08 357014.847715973 -678788.500258861;-0.00064 8.75621643227654e-08 367209.789786894 -673327.861276952;-0.0006 8.7501761643589e-08 377321.231518299 -667714.113345921;-0.00056 8.74214618183979e-08 387346.873655537 -661948.532983636;-0.00052 8.73212831066798e-08 397284.436454043 -656032.431233352;-0.00048 8.720124828821e-08 407131.660197734 -649967.153365589;-0.00044 8.7061384657871e-08 416886.30571285 -643754.078572227;-0.0004 8.69017240194462e-08 426546.154877121 -637394.619652898;-0.00036 8.67223026783879e-08 436109.011124151 -630890.222693716;-0.00032 8.65231614335618e-08 445572.699942895 -624242.366738459;-0.00028 8.63043455679697e-08 454935.069372127 -617452.563452243;-0.00024 8.60659048384524e-08 464193.990489777 -610522.356777782;-0.0002 8.58078934643757e-08 473347.357897028 -603453.322584311;-0.00016 8.55303701153008e-08 482393.090197068 -596247.068309243;-0.00012 8.52333978976443e-08 491329.130468377 -588905.232592658;-8e-05 8.49170443403273e-08 500153.446732459 -581429.484904683;-4e-05 8.45813813794208e-08 508864.032415895 -573821.525165876]  x2=[-0.00136 1.45974070409112e-07 0 0;-0.00132 1.4650256590852e-07 0 0;-0.00128 1.46997747987825e-07 0 0;-0.00124 1.47459504046892e-07 0 0;-0.0012 1.47887729086375e-07 0 0;-0.00116 1.48282325731594e-07 0 0;-0.00112 1.48643204254673e-07 0 0;-0.00108 1.4897028259495e-07 0 0;-0.00104 1.49263486377629e-07 0 0;-0.001 1.49522748930699e-07 0 0;-0.00096 1.49748011300092e-07 0 0;-0.00092 1.49939222263087e-07 0 0;-0.00088 1.50096338339961e-07 0 0;-0.00084 1.50219323803871e-07 177817.551288418 -753238.639328539;-0.0008 1.50308150688985e-07 189155.50082339 -750471.655165856;-0.00076 1.50362798796834e-07 200450.438028681 -747534.02022058;-0.00072 1.50383255700911e-07 211699.794532977 -744426.402485564;-0.00068 1.50369516749491e-07 222901.012329616 -741149.508606283;-0.00064 1.50321585066693e-07 234051.544358269 -737704.083720146;-0.0006 1.5023947155177e-07 245148.855084109 -734090.91128706;-0.00056 1.50123194876626e-07 256190.421074376 -730310.812911278;-0.00052 1.49972781481574e-07 267173.731572183 -726364.648154572;-0.00048 1.49788265569324e-07 278096.289067439 -722253.314340778;-0.00044 1.49569689097202e-07 288955.609864761 -717977.74635175;-0.0004 1.49317101767613e-07 299749.224648247 -713538.916414778;-0.00036 1.49030561016738e-07 310474.679042975 -708937.83388151;-0.00032 1.48710132001473e-07 321129.534173109 -704175.544998438;-0.00028 1.48355887584612e-07 331711.367216474 -699253.132668984;-0.00024 1.47967908318282e-07 342217.771955492 -694171.716207264;-0.0002 1.4754628242562e-07 352646.359324327 -688932.45108356;-0.00016 1.4709110578072e-07 362994.757952144 -683536.528661579;-0.00012 1.46602481886825e-07 373260.614702337 -677985.17592755;-8e-05 1.46080521852795e-07 383441.595207609 -672279.655211209;-4e-05 1.45525344367841e-07 393535.38440079 -666421.263898766]  x3=[-0.00136 5.74670784517293e-10 0 0;-0.00132 5.94260294069406e-10 0 0;-0.00128 6.13714673955329e-10 0 0;-0.00124 6.33029500416845e-10 0 0;-0.0012 6.5220038142898e-10 0 0;-0.00116 6.71222957698714e-10 0 0;-0.00112 6.90092903656248e-10 0 0;-0.00108 7.08805928438599e-10 0 0;-0.00104 7.27357776865304e-10 0 0;-0.001 7.45744230406017e-10 0 0;-0.00096 7.6396110813976e-10 0 0;-0.00092 7.82004267705632e-10 0 0;-0.00088 7.99869606244744e-10 0 0;-0.00084 8.17553061333179e-10 247.5796802977 -6549.91554754019;-0.0008 8.35050611905744e-10 346.318244179341 -6545.43753477073;-0.00076 8.52358279170331e-10 444.978058278777 -6539.47114595132;-0.00072 8.6947212751266e-10 543.536688205088 -6532.01773778732;-0.00068 8.863882653912e-10 641.971722575762 -6523.07900511947;-0.00064 9.03102846222078e-10 740.260778112851 -6512.65698053849;-0.0006 9.19612069253752e-10 838.381504732734 -6500.75403392289;-0.00056 9.35912180431274e-10 936.311590628334 -6487.3728719001;-0.00052 9.51999473249929e-10 1034.02876734263 -6472.51653723096;-0.00048 9.67870289598061e-10 1131.51081483232 -6456.18840811786;-0.00044 9.83521020588896e-10 1228.73556652045 -6438.39219743655;-0.0004 9.98948107381173e-10 1325.68091433692 -6419.13195189187;-0.00036 1.01414804198839e-09 1422.32481374565 -6398.41205109756;-0.00032 1.02911736807651e-09 1518.64528875735 -6376.2372065804;-0.00028 1.04385268174985e-09 1614.62043692662 -6352.61246070878;-0.00024 1.05835063232516e-09 1710.22843433242 -6327.5431855462;-0.0002 1.07260792309351e-09 1805.44754054065 -6301.03508162963;-0.00016 1.08662131206993e-09 1900.25610354766 -6273.09417667331;-0.00012 1.1003876127306e-09 1994.63256470385 -6243.72682419808;-8e-05 1.11390369473748e-09 2088.55546361579 -6212.93970208663;-4e-05 1.12716648465007e-09 2182.00344302625 -6180.73981106504]  x4=[-0.00136 1.04097843869864e-09 0 0;-0.00132 1.03461627691198e-09 0 0;-0.00128 1.02801885230609e-09 0 0;-0.00124 1.02118766507845e-09 0 0;-0.0012 1.01412426858212e-09 0 0;-0.00116 1.00683026897254e-09 0 0;-0.00112 9.99307324842342e-10 0 0;-0.00108 9.91557146844129e-10 0 0;-0.00104 9.83581497301549e-10 0 0;-0.001 9.75382189808527e-10 0 0;-0.00096 9.66961088816881e-10 0 0;-0.00092 9.58320109212356e-10 0 0;-0.00088 9.49461215879196e-10 0 0;-0.00084 9.4038642325335e-10 5643.35735450968 -27050.4610325523;-0.0008 9.31097794864403e-10 6050.61269513804 -26962.2880413409;-0.00076 9.2159744286635e-10 6456.49217861779 -26867.9840583416;-0.00072 9.11887527557306e-10 6860.90351145455 -26767.5705274672;-0.00068 9.0197025688828e-10 7263.7547339987 -26661.0702818885;-0.00064 8.91847885961097e-10 7664.95424135631 -26548.507538843;-0.0006 8.81522716515615e-10 8064.41080421917 -26429.9078941277;-0.00056 8.70997096406325e-10 8462.03358960967 -26305.2983162791;-0.00052 8.60273419068472e-10 8857.73218153537 -26174.7071404407;-0.00048 8.49354122973805e-10 9251.41660154882 -26038.1640619195;-0.00044 8.38241691076091e-10 9642.99732920789 -25895.7001294342;-0.0004 8.26938650246515e-10 10032.385322432 -25747.3477380546;-0.00036 8.15447570699089e-10 10419.4920377493 -25593.1406218349;-0.00032 8.03771065406206e-10 10804.2294504312 -25433.1138461437;-0.00028 7.91911789504475e-10 11186.5100745077 -25267.3037996897;-0.00024 7.79872439690968e-10 11566.2469826616 -25095.7481862476;-0.0002 7.67655753610009e-10 11943.3538259948 -24918.4860160845;-0.00016 7.5526450923066e-10 12317.744853663 -24735.5575970891;-0.00012 7.42701524215036e-10 12689.3349323752 -24547.0045256066;-8e-05 7.2996965527759e-10 13058.0395657519 -24352.8696769793;-4e-05 7.17071797535524e-10 13423.7749135392 -24153.1971957977]  x5=0.00133467809810995  V1=ones(3,3)  V2=ones(3,3)  I1=ones(3,3)  I2=ones(3,3)  nHarmo=1  Measurements=None  Decoupling=off  VsMag0=0  VrMag0=0  VsAngle0=0  VrAngle0=0  IsMag0=0  IrMag0=0  IsAngle0=0  IrAngle0=0
      settings: AttributesFormatString=\n
  NEM-ALB 1980 Mvar : powerlib/Elements/Three-Phase Series RLC Load  LConnTagsString=A|B|C  Configuration=Y (grounded)  NominalVoltage=735e3  Vabc=[1e3 1e3 1e3]  Vabcp=[1e3 1e3 1e3]  NominalFrequency=60  UnbalancedPower=off  ActivePower=6600000  InductivePower=1980e6  CapacitivePower=0  Pabc=[10e3 9e3 11e3]  QLabc=[100 90 110]  QCabc=[100 90 110]  Pabcp=[10e3 9e3 11e3]  QLabcp=[100 90 110]  QCabcp=[100 90 110]  Measurements=None  LoadType=constant Z
  NEM-ALB7 : powerlib/Measurements/Three-Phase V-I Measurement  VoltageMeasurement=no  SetLabelV=on  LabelV=Vabc_NEM7  Vpu=on  VpuLL=off  CurrentMeasurement=no  SetLabelI=off  LabelI=A1  Ipu=off  Pbase=100e6  Vbase=735e3  OutputType=Magnitude  PhasorSimulation=off  PSBequivalent=0
  Regulators1 : Subsystem
  Regulators2 : Subsystem
  Regulators3 : Subsystem
  Regulators4 : Subsystem
  MTLa : PMIOPort  Side=Right
  MTLb : PMIOPort  Port=2  Side=Right
  MTLc : PMIOPort  Port=3  Side=Right
  CHM7a : PMIOPort  Port=4  Side=Right
  CHM7b : PMIOPort  Port=5  Side=Right
  CHM7c : PMIOPort  Port=6  Side=Right
  wires:
  Regulators2/1(Pm) -> LG3_2200 MVA/1
  Regulators4/2(Vf) -> LG4-2700 MVA/2
  Regulators4/1(Pm) -> LG4-2700 MVA/1
  Regulators3/2(Vf) -> LG31-200 MVA/2
  Regulators3/1(Pm) -> LG31-200 MVA/1
  Regulators2/2(Vf) -> LG3_2200 MVA/2
  LG3_2200 MVA/1 -> Regulators2/1(m)
  Regulators1/1(Pm) -> LG2_5500 MVA/1
  Regulators1/2(Vf) -> LG2_5500 MVA/2
  LG2_5500 MVA/1 -> Regulators1/1(m)
  LG31-200 MVA/1 -> Regulators3/1(m)
  LG4-2700 MVA/1 -> Regulators4/1(m)
  connections:
  LG2-NENI 3*279km/RConn1 -- "Cs NEM "/LConn1
  LG2-NENI 3*279km/RConn2 -- "Cs NEM "/LConn2
  LG2-NENI 3*279km/RConn3 -- "Cs NEM "/LConn3
  CHB-CHM 3*195km/RConn1 -- "Cs  CHMN "/LConn1
  CHB-CHM 3*195km/RConn2 -- "Cs  CHMN "/LConn2
  CHB-CHM 3*195km/RConn3 -- "Cs  CHMN "/LConn3
  Load Flow Bus2/LConn1 -- 2200 MVA 13.8 kV/735 kV/LConn1 -- LG3_2200 MVA/RConn1 -- 110 MW/LConn1
  2200 MVA 13.8 kV/735 kV/LConn2 -- LG3_2200 MVA/RConn2 -- 110 MW/LConn2
  2200 MVA 13.8 kV/735 kV/LConn3 -- LG3_2200 MVA/RConn3 -- 110 MW/LConn3
  Load Flow Bus1/LConn1 -- 200 MVA 13.8 kV/735 kV/LConn1 -- LG31-200 MVA/RConn1 -- 10 MW/LConn1
  200 MVA 13.8 kV/735 kV/LConn2 -- LG31-200 MVA/RConn2 -- 10 MW/LConn2
  200 MVA 13.8 kV/735 kV/LConn3 -- LG31-200 MVA/RConn3 -- 10 MW/LConn3
  Load Flow Bus6/LConn1 -- 2200 MVA 13.8 kV/735 kV/RConn1 -- 200 MVA 13.8 kV/735 kV/RConn1 -- LG3-LMO 104km/LConn1 -- LG3 660 Mvar/LConn1 -- LG2-LG3 155km/RConn1
  2200 MVA 13.8 kV/735 kV/RConn2 -- LG3 660 Mvar/LConn2 -- LG2-LG3 155km/RConn2 -- 200 MVA 13.8 kV/735 kV/RConn2 -- LG3-LMO 104km/LConn2
  LG3-LMO 104km/RConn1 -- LMO7/RConn1 -- LG4-LMO 3*118km/RConn1 -- LMO 330 Mvar/LConn1
  LG3-LMO 104km/RConn2 -- LMO7/RConn2 -- LG4-LMO 3*118km/RConn2 -- LMO 330 Mvar/LConn2
  LG3-LMO 104km/RConn3 -- LMO7/RConn3 -- LG4-LMO 3*118km/RConn3 -- LMO 330 Mvar/LConn3
  LG4-LMO 3*118km/LConn1 -- LG4 660 Mvar/LConn1 -- 2700 MVA 13.8 kV/735 kV/RConn1 -- Load Flow Bus12/LConn1
  LG4-LMO 3*118km/LConn2 -- 2700 MVA 13.8 kV/735 kV/RConn2 -- LG4 660 Mvar/LConn2
  LG4 660 Mvar/LConn3 -- 2700 MVA 13.8 kV/735 kV/RConn3 -- LG4-LMO 3*118km/LConn3
  Load Flow Bus3/LConn1 -- LG4-2700 MVA/RConn1 -- 2700 MVA 13.8 kV/735 kV/LConn1 -- 135 MW/LConn1
  LG4-2700 MVA/RConn2 -- 2700 MVA 13.8 kV/735 kV/LConn2 -- 135 MW/LConn2
  LG4-2700 MVA/RConn3 -- 2700 MVA 13.8 kV/735 kV/LConn3 -- 135 MW/LConn3
  Load Flow Bus4/LConn1 -- 5500 MVA 13.8 kV/735 kV/LConn1 -- LG2_5500 MVA/RConn1 -- 275 MW/LConn1
  5500 MVA 13.8 kV/735 kV/LConn2 -- LG2_5500 MVA/RConn2 -- 275 MW/LConn2
  LG2_5500 MVA/RConn3 -- 5500 MVA 13.8 kV/735 kV/LConn3 -- 275 MW/LConn3
  5500 MVA 13.8 kV/735 kV/RConn1 -- LG2-NENI 3*279km/LConn1 -- LG2-LG3 155km/LConn1 -- LG2 660 Mvar/LConn1 -- Load Flow Bus5/LConn1
  LG2-LG3 155km/LConn2 -- 5500 MVA 13.8 kV/735 kV/RConn2 -- LG2-NENI 3*279km/LConn2 -- LG2 660 Mvar/LConn2
  LG2-LG3 155km/LConn3 -- 5500 MVA 13.8 kV/735 kV/RConn3 -- LG2-NENI 3*279km/LConn3 -- LG2 660 Mvar/LConn3
  "Cs NEM "/RConn1 -- NEM-ALB7/LConn1 -- Cs ALB/RConn1
  "Cs NEM "/RConn2 -- NEM-ALB7/LConn2 -- Cs ALB/RConn2
  "Cs NEM "/RConn3 -- NEM-ALB7/LConn3 -- Cs ALB/RConn3
  LMO7/LConn1 -- LMO-ALB 3*218km/LConn1
  LMO7/LConn2 -- LMO-ALB 3*218km/LConn2
  Load Flow Bus7/LConn1 -- LMO7/LConn3 -- LMO-ALB 3*218km/LConn3
  Cs ALB/LConn1 -- LMO-ALB 3*218km/RConn1
  Cs ALB/LConn2 -- LMO-ALB 3*218km/RConn2
  Cs ALB/LConn3 -- LMO-ALB 3*218km/RConn3
  200 MVA 13.8 kV/735 kV/RConn3 -- LG3-LMO 104km/LConn3 -- LG3 660 Mvar/LConn3 -- LG2-LG3 155km/RConn3 -- 2200 MVA 13.8 kV/735 kV/RConn3
  Load Flow Bus8/LConn1 -- NEM-ABI 6*236/LConn1 -- NEM-ALB7/RConn1 -- NEM-ALB 1980 Mvar/LConn1
  NEM-ALB 1980 Mvar/LConn2 -- NEM-ALB7/RConn2 -- NEM-ABI 6*236/LConn2
  NEM-ALB 1980 Mvar/LConn3 -- NEM-ALB7/RConn3 -- NEM-ABI 6*236/LConn3
  NEM-ABI 6*236/RConn1 -- "Cs ABI+CHB "/LConn1
  NEM-ABI 6*236/RConn2 -- "Cs ABI+CHB "/LConn2
  NEM-ABI 6*236/RConn3 -- "Cs ABI+CHB "/LConn3
  "Cs ABI+CHB "/RConn1 -- ABI-CHB7/LConn1
  "Cs ABI+CHB "/RConn2 -- ABI-CHB7/LConn2
  "Cs ABI+CHB "/RConn3 -- ABI-CHB7/LConn3
  Load Flow Bus9/LConn1 -- ABI+CHB 1320 Mvar/LConn1 -- CHB-CHM 3*195km/LConn1 -- ABI-CHB 3*271km/LConn1 -- ABI-CHB7/RConn1
  ABI-CHB 3*271km/LConn2 -- ABI-CHB7/RConn2 -- ABI+CHB 1320 Mvar/LConn2 -- CHB-CHM 3*195km/LConn2
  ABI-CHB 3*271km/LConn3 -- ABI-CHB7/RConn3 -- ABI+CHB 1320 Mvar/LConn3 -- CHB-CHM 3*195km/LConn3
  ABI-CHB 3*271km/RConn1 -- "Cs LVDN "/LConn1
  ABI-CHB 3*271km/RConn2 -- "Cs LVDN "/LConn2
  ABI-CHB 3*271km/RConn3 -- "Cs LVDN "/LConn3
  "Cs LVDN "/RConn1 -- LVD7/LConn1
  "Cs LVDN "/RConn2 -- LVD7/LConn2
  "Cs LVDN "/RConn3 -- LVD7/LConn3
  "Cs LVDS "/LConn1 -- LVD 990 Mvar/LConn1 -- Load Flow Bus10/LConn1 -- LVD7/RConn1
  "Cs LVDS "/LConn2 -- LVD7/RConn2 -- LVD 990 Mvar/LConn2
  "Cs LVDS "/LConn3 -- LVD7/RConn3 -- LVD 990 Mvar/LConn3
  "Cs LVDS "/RConn1 -- LVD-MTL 3*260km/LConn1
  "Cs LVDS "/RConn2 -- LVD-MTL 3*260km/LConn2
  "Cs LVDS "/RConn3 -- LVD-MTL 3*260km/LConn3
  MTLa/RConn1 -- LVD-MTL 3*260km/RConn1
  MTLb/RConn1 -- LVD-MTL 3*260km/RConn2
  MTLc/RConn1 -- LVD-MTL 3*260km/RConn3
  "Cs  CHMN "/RConn1 -- CHM7/LConn1
  "Cs  CHMN "/RConn2 -- CHM7/LConn2
  "Cs  CHMN "/RConn3 -- CHM7/LConn3
  CHM 1320Mvar/LConn2 -- CHM7/RConn2 -- CHM7b/RConn1
  Load Flow Bus11/LConn1 -- CHM 1320Mvar/LConn3 -- CHM7c/RConn1 -- CHM7/RConn3
  CHM7a/RConn1 -- CHM 1320Mvar/LConn1 -- CHM7/RConn1
